simulink library "vmc"  (R2021b)
settings: Solver=VariableStepAuto  StartTime=0.0  StopTime=10.0  RelTol=1e-3
undefined symbols (not defined in the file): AVMC_ACCDeltaTqGradeGn_X_deg, AVMC_ACCDeltaTqIGain4OVRD_X_kph, AVMC_ACCDeltaTqIGain4OVRD_Y_mps2, AVMC_ACCDeltaTqIGain_X_kph, AVMC_ACCDeltaTqIGain_Y_mps2, AVMC_ACCDeltaTqPGain_X_kph, AVMC_ACCDeltaTqPGain_Y_kph, AVMC_ACCGradeofst_X_G, AVMC_ACCGradeofst_Y_pct, AVMC_ACCLoSpdTqLoLim4JP_X_kph, AVMC_ACCLoSpdTqLoLim4JP_Y_deg, AVMC_ACCLoSpdTqLowerLim_X_kph, AVMC_ACCLoSpdTqLowerLim_Y_deg, AVMC_ACCReqAccelGain_X_mps2, AVMC_ACCReqAccelGain_Y_enum, AVMC_ADSPosGFBDeltaTq_X_kph, AVMC_ADSPosGFBDeltaTq_Y_mps2, AVMC_AggressJerkPCT4AT_X_kph, AVMC_AggressJerkPCT_X_kph, AVMC_AggressLimitPCT4AT_X_kph, AVMC_AggressLimitPCT_X_kph, AVMC_DECGradeofst_X_G, AVMC_DECGradeofst_Y_pct, AVMC_DISCDeltaTqIGain_X_kph, AVMC_DISCDeltaTqIGain_Y_mps2, AVMC_DISCDeltaTqPGain_X_kph, AVMC_DISCDeltaTqPGain_Y_kph, AVMC_EPSForceSelect_X_enum, AVMC_EPSForceSelect_Y_enum, AVMC_EPSForceSelectD21_X_enum, AVMC_EPSForceSelectD21_Y_enum, AVMC_ESCRegenOut_X_kph, AVMC_ESCRegenOut_Y_Deg, AVMC_ESCRegenOutEnSpd_X_Deg, AVMC_EstPitchSlopeTs_X_kph, AVMC_GradeCompFlt_X_kph, AVMC_GyroYBandLo_X_Gps, AVMC_HoldResTq_X_kph, AVMC_ISOAccLimit_X_mps, AVMC_ISODecLimit_X_mps, AVMC_ISOJerk_X_mps, AVMC_LatESCRegenOut_X_kph, AVMC_LatESCRegenOut_Y_Deg, AVMC_LongAccDeadZone_X_kph, AVMC_LongAccFiltTsforP2_X_Gps, AVMC_MCPresBaseTq_X_bar, AVMC_MSAPedalOvrd_X_kph, AVMC_MSASpdBand_X_kph, AVMC_MSATqDownEndTq_X_kph, AVMC_MSATqDownTime_X_kph, AVMC_NegZCHoldTq_X_kph, AVMC_OPDDisSlideRate_X_Deg, AVMC_OVRD2ActSR2FCMCMD_X_mps2, AVMC_PedalTqRWhlRatio_X_Nm, AVMC_PedalTqRWhlRatio_Y_gps, AVMC_PedalTqRWhlSlipGain_X_rat, AVMC_PedalTqRWhlSlipGain_Y_kph, AVMC_PedalTqRWhSTRGGain_X_deg, AVMC_PedalTqRWhSTRGGain_Y_kph, AVMC_PosZCHoldTq_X_kph ... (+593)
libraries: hcu_lib x143, simulink x96, tqr x4, $bdroot x1, simulink_extras x1
(part 8 of 17)

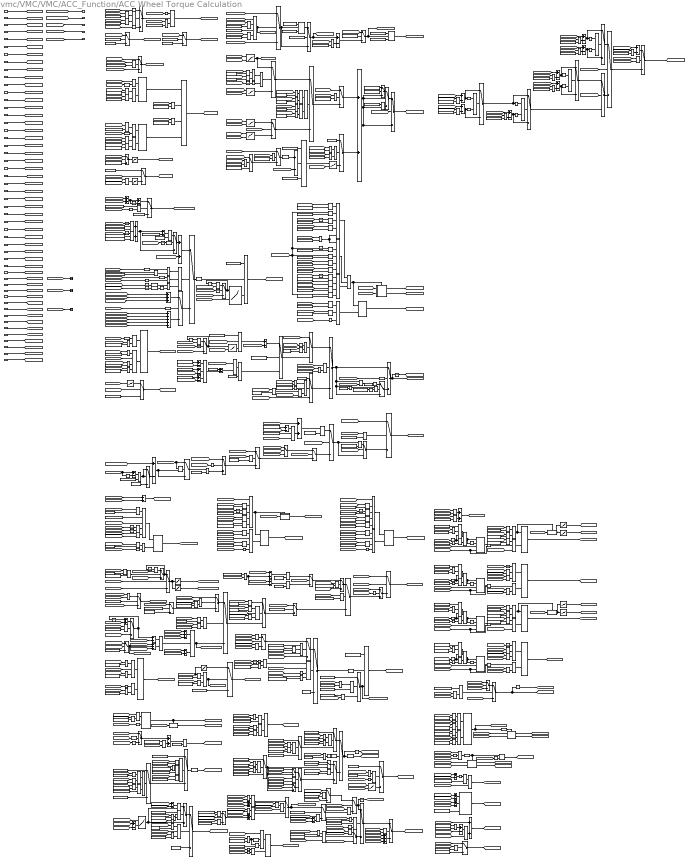
== system vmc/VMC/VMC/ACC_Function/ACC Wheel Torque Calculation ==
  note: HoldTqCalculation
  note: ZeroCrossControl
  note: VehHoldJerkPrevent
  note: ADASWhlTqCalAftHold_ADASWhlTqReq
  note: ADASWhlTqCalBftHold
  note: OriADASWhlTq_ACCLowSpdTq
  note: ACCDeltaTq
  note: GradeHoldResumeAddTq
  note: NegReq_BRgn_TqCompensation
  note: Deceleration Positive Torque Control
  note: Deceleration Torque Control
  note: Deceleration REGEN Torque Control Judgement
  note: Deceleration REGEN Torque Control
  VVMC_LongAcc_Gps : Inport
  VVMC_ActACCRequiredAccel_mps2 : Inport  Port=2
  VVMC_VehicleSpeed_kph : Inport  Port=3
  VVMC_ADASActive_flg : Inport  Port=4
  VTQD_CoordWhlTqDemFr_Nm : Inport  Port=5
  VTQD_CoordWhlTqDemRr_Nm : Inport  Port=6
  VVMC_ACCPedalOvrd_flg : Inport  Port=7
  VVMC_FeatSetSpdForCalcu_kph : Inport  Port=8
  VVMC_FeatArbitrFinal_enum : Inport  Port=9
  VINP_FrTMSpd_rpm : Inport  Port=10
  VINP_RrTMSpd_rpm : Inport  Port=11
  VINP_MCPressure_bar : Inport  Port=12
  VINP_ESCADASSta_enum : Inport  Port=13
  VVMC_FeatReqSpd_kph : Inport  Port=14
  VVMC_MeterIndSpeedForCalcu_kph : Inport  Port=15
  VTQD_SWC2ResUpSta_flg : Inport  Port=16
  VINP_FrntAxlTrqReqBrk_Nm : Inport  Port=17
  VINP_RearAxlTrqReqBrk_Nm : Inport  Port=18
  VTQR_RrTMTqReq_Nm : Inport  Port=19
  VVMC_ACCVehHoldReqRaw_flg : Inport  Port=20
  VVMC_EstSlope_Deg : Inport  Port=21
  VINP_TargetType_enum : Inport  Port=22
  VVMC_SafetyCtrl_flg : Inport  Port=23
  VTQR_FrTMTqReq_Nm : Inport  Port=24
  task_time_s : Inport  Port=25
  VVMC_TotalAvailBrkRgnTq_Nm : Inport  Port=26
  VVMC_AccelTurnHold_flg : Inport  Port=27
  VVMC_ADASACCSta_enum : Inport  Port=28
  VTQD_CreepBaseTqD_Nm : Inport  Port=29
  VVMC_OVRD2ActRampActive_flg : Inport  Port=30
  VINP_ACCRequiredAccel_mps2 : Inport  Port=31
  VTQD_SWC1ResUpSta_flg : Inport  Port=32
  VINP_SWCType_enum : Inport  Port=33
  VVMC_ReqBrkJoin_flg : Inport  Port=34
  VINP_RDCActive_enum : Inport  Port=35
  VINP_BrkSwSta_flg : Inport  Port=36
  VINP_LFWhlRotDir_enum : Inport  Port=37
  VINP_LRWhlRotDir_enum : Inport  Port=38
  VINP_RFWhlRotDir_enum : Inport  Port=39
  VINP_RRWhlRotDir_enum : Inport  Port=40
  VINP_FrEDURealTMTq_Nm : Inport  Port=41
  VINP_FrEDURotateDirction_enum : Inport  Port=42
  VINP_RrEDURealTMTq_Nm : Inport  Port=43
  VINP_RrEDURotateDirction_enum : Inport  Port=44
  VVMC_ACCVehHoldReq_flg : Inport  Port=45
  VVMC_ACCShutOffHold_flg : Inport  Port=46
  VVMC_FrWhlSpdInvalid_flg : Inport  Port=47
  VVMC_RrWhlSpdInvalid_flg : Inport  Port=48
  VVMC_LongAccFrWhl_Gps : Inport  Port=49
  VVMC_LongAccRrWhl_Gps : Inport  Port=50
  " 2" : Constant  Value=ENUM_SWCTYPE_SWC2
  1-D Lookup Table : Lookup_n-D  NumberOfTableDimensions=1  BreakpointsForDimension1=AVMC_ACCDeltaTqGradeGn_X_deg  Table=MVMC_ACCDeltaTqGradeGn_Y_Nm  InternalRulePriority=Speed  RndMeth=Simplest  InputSameDT=on
  AND{,1,4,7..8,10..11,16..18,20..27,31..33,38,41,44,47..49,52..53,55,60,62} (32 alike) : Logic  AllPortsSameDT=off  OutDataTypeStr=boolean
  AND{2,6,12..13,28..30,34,36,39,42,45,50..51,54,56..57,61} (18 alike) : Logic  Inputs=3  AllPortsSameDT=off  OutDataTypeStr=boolean
  AND{14..15,19,35,37,40,43,46} (8 alike) : Logic  Operator=OR  AllPortsSameDT=off  OutDataTypeStr=boolean
  AND3 : Logic  Inputs=4  AllPortsSameDT=off  OutDataTypeStr=boolean
  AND5 : Logic  Inputs=5  AllPortsSameDT=off  OutDataTypeStr=boolean
  AND58 : Logic  Operator=OR  Inputs=3  AllPortsSameDT=off  OutDataTypeStr=boolean
  AND59 : Logic  Operator=OR  Inputs=4  AllPortsSameDT=off  OutDataTypeStr=boolean
  AND9 : Logic  Inputs=4  AllPortsSameDT=off  OutDataTypeStr=boolean
  Abs{,1..8} (9 alike) : Abs
  Add{,3..4,7..8,10..12,14,16,27,30..35,40..46,48} (25 alike) : Sum  Inputs=+-
  Add1 : Sum  Inputs=+++++
  Add{2,5..6,13,15,18..21,23,25..26,28..29,36..39} (18 alike) : Sum
  Add{9,17,22,24} (4 alike) : Sum  Inputs=+++
  Cast To Single{,1..3} (4 alike) : DataTypeConversion  OutDataTypeStr=single
  Constant{1,49,76,113,134} (5 alike) : Constant  Value=KVMC_ACCRgnCtrl2Hold_flg
  Constant10 : Constant  Value=KVMC_ADASWhlTqUpperLim_Nm
  Constant100 : Constant  Value=KVMC_ZeroRgnTqSpdCtrlTime_s
  Constant{4,18..19,22,25,27,29,40,43,45..46,50..53,58,63..64,66..75,81..83,87,89..90,92..94,96,98..99,101..103,109,111..112,114,116..117,119..120,124..125,129..133,136..137,141..144,151..152,154..156,159,163,168,188,191..192,213,215,219,221,228,234} (81 alike) : Constant  Value=ZERO_FLOAT
  Constant104 : Constant  Value=KVMC_HoldAllowZeroTqGrade_deg
  Constant105 : Constant  Value=KVMC_SmallGradeTMRevPrvt_flg
  Constant106 : Constant  Value=KVMC_VehHoldTqIncMinTq_Nm
  Constant{107..108,208,235} (4 alike) : Constant  Value=KVMC_VehHoldTqIncMCP_bar
  Constant11 : Constant  Value=KVMC_ADASWhlTqLowerLim_Nm
  Constant110 : Constant  Value=KVMC_NegReqEnSpd_kph
  Constant115 : Constant  Value=KVMC_TMRevPrvtTqAddEveryTT_flg
  Constant118 : Constant  Value=KVMC_ACCLoSpdFollowBRgnSW_flg
  Constant12 : Constant  Value=KVMC_AccDevLowLim_mps2
  Constant121 : Constant  Value=KVMC_VHJerkPrvt_flg
  Constant122 : Constant  Value=KVMC_VehHoldDecSR_Nm
  Constant123 : Constant  Value=ENUM_FEATARBITRSTA_DISC
  Constant126 : Constant  Value=KVMC_ADASWhlTqLowerLim_Nm
  Constant127 : Constant  Value=KVMC_VHJerkPrvt_flg
  Constant{41,44,47..48,78..79,91,128,149} (9 alike) : Constant  Value=KVMC_ZeroRgnTqSpd_kph
  Constant13 : Constant  Value=KVMC_AccDevUpLim_mps2
  Constant135 : Constant  Value=KVMC_NegReqDeltaTqGain_rat
  Constant138 : Constant  Value=KVMC_ReqAccelLimitSW_flg
  Constant139 : Constant  Value=KVMC_MaxReqAccel_mps2
  Constant14 : Constant  Value=KVMC_ACCSpdDevUpLim_kph
  Constant140 : Constant  Value=KVMC_MinReqAccel_mps2
  Constant145 : Constant  Value=ENUM_CANRDCACTSTA_EXITIMMEDIATELY
  Constant146 : Constant  Value=KVMC_ADASWhlTqUpperLim_Nm
  Constant147 : Constant  Value=ENUM_CANRDCACTSTA_NOREQUEST
  Constant148 : Constant  Value=KVMC_VHTMSpdCtrlChkTMDir_flg
  Constant15 : Constant  Value=KVMC_ACCSpdDevLowLim_kph
  Constant150 : Constant  Value=KVMC_VHTMSpdCtrlSR_raw32
  Constant153 : Constant  Value=KVMC_ZeroCrossTestSW_flg
  Constant157 : Constant  Value=KTQD_FrTMTotalGearRatio_gain
  Constant158 : Constant  Value=KTQD_RrTMTotalGearRatio_gain
  Constant16 : Constant  Value=ENUM_FEATARBITRSTA_ACC
  Constant160 : Constant  Value=KVMC_VHTMSpdCtrlChkTMDir_flg
  Constant{161..162,171..172,189..190,193..194} (8 alike) : Constant  Value=KVMC_ZCChkRealWhlTqSW_flg
  Constant164 : Constant  Value=KVMC_ESCSSMCPThres_bar
  Constant{165,169..170,173..174,176,184,203..205} (10 alike) : Constant  Value=ENUM_WheelRotDir_BACKWARD
  Constant166 : Constant  Value=ENUM_ESCADASSTA_VEHASTANDSTILL
  Constant167 : Constant  Value=KVMC_StandstillTqRamp2ZeroSlope_Nmps
  Constant{17,211,224,226,232} (5 alike) : Constant  Value=ENUM_ADASACCSTA_ACTIVE
  Constant{175,177..178,181,197,206} (6 alike) : Constant  Value=ENUM_WheelRotDir_FORWARD
  Constant{179..180,182..183,185..187,198,200} (9 alike) : Constant  Value=ENUM_WheelRotDir_STANDSTILL
  Constant195 : Constant  Value=ENUM_TMROTATEDIRECTACT_STOP
  Constant196 : Constant  Value=ENUM_TMROTATEDIRECTACT_REVERSE
  Constant199 : Constant  Value=KVMC_HoldAdd2GradeGn_flg
  Constant{2,7..8,20} (4 alike) : Constant  Value=KVMC_HillUpResetTMSpd_rpm
  Constant201 : Constant  Value=KVMC_VHTMSpdCtrlChkTMDir_flg
  Constant202 : Constant  Value=ENUM_TMROTATEDIRECTACT_STOP
  Constant207 : Constant  Value=KVMC_IgnrAvailBrgnSpd_kph
  Constant209 : Constant  Value=KVMC_HoldTqCalSpd1_kph
  Constant21 : Constant  Value=ENUM_FEATARBITRSTA_DISC
  Constant{9,210,229,237..243,245} (11 alike) : Constant  Value=KVMC_GravityValue_mps2
  Constant212 : Constant  Value=KVMC_HoldTqCalDeltaAccThres_Gps
  Constant214 : Constant  Value=KVMC_HoldTqCtrlTargetGx_mps2
  Constant{216..218,223} (4 alike) : Constant  Value=KVMC_HoldTqCalTest_flg
  Constant220 : Constant  Value=MINUSONE_FLOAT
  Constant222 : Constant  Value=KVMC_AccTurnHoldTqDecSR_Nmps
  Constant225 : Constant  Value=KVMC_HoldTqCalSpd1_kph
  Constant227 : Constant  Value=KVMC_HoldGradeOnlyInc_flg
  Constant23 : Constant  Value=KVMC_OVRDResSmoothTest_SW
  Constant230 : Constant  Value=KVMC_HoldTqAddDisDec_mps2
  Constant231 : Constant  Value=KVMC_HoldResTqDisSpd_kph
  Constant233 : Constant  Value=KVMC_HoldResTqDisDeltaAcc_mps2
  Constant236 : Constant  Value=KVMC_CompareFrRrLongAcl_flg
  Constant24 : Constant  Value=KVMC_OVRD2ActRgnTarget_Nm
  Constant26 : Constant  Value=KVMC_AddBRegen2ACCLoop_flg
  Constant28 : Constant  Value=KVMC_HoldTqCtrlGradeThres_deg
  Constant3 : Constant  Value=ENUM_ESCADASSTA_VEHASTANDSTILL
  Constant30 : Constant  Value=KVMC_TqSafetyCtrl_flg
  Constant31 : Constant  Value=KVMC_ACCResUpEnAccCMD_mps2
  Constant32 : Constant  Value=KVMC_HoldTqCtrlSourceSW_flg
  Constant33 : Constant  Value=KVMC_SoftUphillTqIncSR_Nm
  Constant34 : Constant  Value=KVMC_ADASWhlTqUpperLim_Nm
  Constant35 : Constant  Value=KVMC_NegReqZeroPosTq_flg
  Constant{6,36..37,62,77,80,88,97} (8 alike) : Constant  Value=KVMC_CutOffNegTqSpd_kph
  Constant38 : Constant  Value=KTQR_FrTMGearEff_c
  Constant39 : Constant  Value=KVMC_ACCDeltaTqFollowADSCmd_flg
  Constant42 : Constant  Value=KTQD_FrTMTotalGearRatio_gain
  Constant5 : Constant  Value=KVMC_AddBRegen2ACCLoop_flg
  Constant54 : Constant  Value=KVMC_NegReqSwEnSpd_kph
  Constant55 : Constant  Value=KVMC_NegReqSwEnSlope_Deg
  Constant56 : Constant  Value=KVMC_ACCResUpEnGrade_Deg
  Constant57 : Constant  Value=ENUM_TARGETTYPE_NONE
  Constant59 : Constant  Value=KVMC_TqMCPRelFactor_Nm
  Constant60 : Constant  Value=ENUM_FEATARBITRSTA_ACC
  Constant61 : Constant  Value=ENUM_FEATARBITRSTA_ACC
  Constant65 : Constant  Value=KVMC_TMRevSpdThres_rpm
  Constant84 : Constant  Value=KTQD_RrTMTotalGearRatio_gain
  Constant85 : Constant  Value=KTQR_RrTMGearEff_c
  Constant86 : Constant  Value=KVMC_OVRDResTqDec4Smooth_Nm
  Constant95 : Constant  Value=KVMC_TMRevSpdPassThres_rpm
  Data Type Conversion1 : DataTypeConversion  OutDataTypeStr=single
  Detect Change : simulink/Logic and Bit Operations/Detect Change  vinit=0  OutDataTypeStr=boolean
  Detect Change1 : simulink/Logic and Bit Operations/Detect Change  vinit=0  OutDataTypeStr=boolean
  Detect Decrease{,1..3} (4 alike) : simulink/Logic and Bit Operations/Detect Decrease  vinit=0.0  OutDataTypeStr=boolean
  Detect Increase{,1..8} (9 alike) : simulink/Logic and Bit Operations/Detect Increase  vinit=0.0  OutDataTypeStr=boolean
  Divide : Product  Inputs=*/*
  Divide1 : Product  Inputs=***
  Divide{2,4,6..11} (8 alike) : Product  Inputs=**
  Divide3 : Product  Inputs=*/*
  Divide5 : Product  Inputs=***
  Equal : RelationalOperator  Operator===  OutDataTypeStr=boolean  RndMeth=Simplest
  Equal1 : RelationalOperator  Operator=<=  OutDataTypeStr=boolean  RndMeth=Simplest
  Equal10 : RelationalOperator  Operator===  OutDataTypeStr=boolean  RndMeth=Simplest
  Equal{4,6,8,11} (4 alike) : RelationalOperator  Operator=<  OutDataTypeStr=boolean  RndMeth=Simplest
  Equal{7,9,12,14} (4 alike) : RelationalOperator  Operator=>  OutDataTypeStr=boolean  RndMeth=Simplest
  Equal13 : RelationalOperator  Operator=<=  OutDataTypeStr=boolean  RndMeth=Simplest
  Equal2 : RelationalOperator  Operator=~=  OutDataTypeStr=boolean  RndMeth=Simplest
  Equal3 : RelationalOperator  OutDataTypeStr=boolean  RndMeth=Simplest
  Equal5 : RelationalOperator  OutDataTypeStr=boolean  RndMeth=Simplest
  Logical Operator : Logic  Inputs=4  AllPortsSameDT=off  OutDataTypeStr=boolean
  Logical Operator1 : Logic  Operator=OR  Inputs=3  AllPortsSameDT=off  OutDataTypeStr=boolean
  Logical Operator{2,4,6,8} (4 alike) : Logic  Inputs=5  AllPortsSameDT=off  OutDataTypeStr=boolean
  Logical Operator3 : Logic  Operator=OR  Inputs=3  AllPortsSameDT=off  OutDataTypeStr=boolean
  Logical Operator5 : Logic  AllPortsSameDT=off  OutDataTypeStr=boolean
  Logical Operator7 : Logic  Operator=OR  Inputs=4  AllPortsSameDT=off  OutDataTypeStr=boolean
  Logical Operator9 : Logic  Operator=OR  Inputs=4  AllPortsSameDT=off  OutDataTypeStr=boolean
  MVMC_ACCDeltaTqIGain4OVRD_Z_Nm : Lookup_n-D  BreakpointsForDimension1=AVMC_ACCDeltaTqIGain4OVRD_Y_mps2  BreakpointsForDimension2=AVMC_ACCDeltaTqIGain4OVRD_X_kph  Table=MVMC_ACCDeltaTqIGain4OVRD_Z_Nm  InternalRulePriority=Speed  RndMeth=Simplest  InputSameDT=on
      settings: InputPortMap=u0,u1
  MVMC_ACCDeltaTqIGain_Z_Nm : Lookup_n-D  BreakpointsForDimension1=AVMC_ACCDeltaTqIGain_Y_mps2  BreakpointsForDimension2=AVMC_ACCDeltaTqIGain_X_kph  Table=MVMC_ACCDeltaTqIGain_Z_Nm  InternalRulePriority=Speed  RndMeth=Simplest  InputSameDT=on
      settings: InputPortMap=u0,u1
  MVMC_ACCDeltaTqPGain_Z_Nm1 : Lookup_n-D  BreakpointsForDimension1=AVMC_ACCDeltaTqPGain_Y_kph  BreakpointsForDimension2=AVMC_ACCDeltaTqPGain_X_kph  Table=MVMC_ACCDeltaTqPGain_Z_Nm  InternalRulePriority=Speed  RndMeth=Simplest  InputSameDT=on
      settings: InputPortMap=u0,u1
  MVMC_ACCLoSpdTqLoLim4JP_Z_Nm : Lookup_n-D  BreakpointsForDimension1=AVMC_ACCLoSpdTqLoLim4JP_Y_deg  BreakpointsForDimension2=AVMC_ACCLoSpdTqLoLim4JP_X_kph  Table=MVMC_ACCLoSpdTqLoLim4JP_Z_Nm  InternalRulePriority=Speed  RndMeth=Simplest  InputSameDT=on
      settings: InputPortMap=u0,u1
  MVMC_ACCLoSpdTqLowerLim_Z_Nm : Lookup_n-D  BreakpointsForDimension1=AVMC_ACCLoSpdTqLowerLim_Y_deg  BreakpointsForDimension2=AVMC_ACCLoSpdTqLowerLim_X_kph  Table=MVMC_ACCLoSpdTqLowerLim_Z_Nm  InternalRulePriority=Speed  RndMeth=Simplest  InputSameDT=on
      settings: InputPortMap=u0,u1
  MVMC_ADSPosGFBDeltaTq_Z_Nm1 : Lookup_n-D  BreakpointsForDimension1=AVMC_ADSPosGFBDeltaTq_Y_mps2  BreakpointsForDimension2=AVMC_ADSPosGFBDeltaTq_X_kph  Table=MVMC_ADSPosGFBDeltaTq_Z_Nm  InternalRulePriority=Speed  RndMeth=Simplest  InputSameDT=on
      settings: InputPortMap=u0,u1
  MVMC_DISCDeltaTqIGain_Z_Nm : Lookup_n-D  BreakpointsForDimension1=AVMC_DISCDeltaTqIGain_Y_mps2  BreakpointsForDimension2=AVMC_DISCDeltaTqIGain_X_kph  Table=MVMC_DISCDeltaTqIGain_Z_Nm  InternalRulePriority=Speed  RndMeth=Simplest  InputSameDT=on
      settings: InputPortMap=u0,u1
  MVMC_HoldResTq_Y_Nm : Lookup_n-D  NumberOfTableDimensions=1  BreakpointsForDimension1=AVMC_HoldResTq_X_kph  Table=MVMC_HoldResTq_Y_Nm  InternalRulePriority=Speed  RndMeth=Simplest  InputSameDT=on
  MVMC_MCPresBaseTq_Y_Nm : Lookup_n-D  NumberOfTableDimensions=1  BreakpointsForDimension1=AVMC_MCPresBaseTq_X_bar  Table=MVMC_MCPresBaseTq_Y_Nm  InternalRulePriority=Speed  RndMeth=Simplest  InputSameDT=on
  MVMC_NegZCHoldTq_Y_Nm : Lookup_n-D  NumberOfTableDimensions=1  BreakpointsForDimension1=AVMC_NegZCHoldTq_X_kph  Table=MVMC_NegZCHoldTq_Y_Nm  InternalRulePriority=Speed  RndMeth=Simplest  InputSameDT=on
  MVMC_PosZCHoldTq_Y_Nm : Lookup_n-D  NumberOfTableDimensions=1  BreakpointsForDimension1=AVMC_PosZCHoldTq_X_kph  Table=MVMC_PosZCHoldTq_Y_Nm  InternalRulePriority=Speed  RndMeth=Simplest  InputSameDT=on
  MVMC_TMRevPrvtTq4JP_Z_Nm : Lookup_n-D  BreakpointsForDimension1=AVMC_TMRevPrvtTq4JP_Y_enum  BreakpointsForDimension2=AVMC_TMRevPrvtTq4JP_X_rpm  Table=MVMC_TMRevPrvtTq4JP_Z_Nm  InternalRulePriority=Speed  RndMeth=Simplest  InputSameDT=on
      settings: InputPortMap=u0,u1
  MVMC_TMRevPrvtTq_Y_Nm : Lookup_n-D  NumberOfTableDimensions=1  BreakpointsForDimension1=AVMC_TMRevPrvtTq_X_rpm  Table=MVMC_TMRevPrvtTq_Y_Nm  InternalRulePriority=Speed  RndMeth=Simplest  InputSameDT=on
  MVMC_TMSpdBaseTq_Y_Nm : Lookup_n-D  NumberOfTableDimensions=1  BreakpointsForDimension1=AVMC_TMSpdBaseTq_X_rpm  Table=MVMC_TMSpdBaseTq_Y_Nm  InternalRulePriority=Speed  RndMeth=Simplest  InputSameDT=on
  MVMC_VHTMSpdCtrl_Z_Nm : Lookup_n-D  BreakpointsForDimension1=AVMC_VHTMSpdCtrl_Y_enum  BreakpointsForDimension2=AVMC_VHTMSpdCtrl_X_rpm  Table=MVMC_VHTMSpdCtrl_Z_Nm  InternalRulePriority=Speed  RndMeth=Simplest  InputSameDT=on
      settings: InputPortMap=u0,u1
  MVMC_VehHoldTqIncGain_Y_Nm : Lookup_n-D  NumberOfTableDimensions=1  BreakpointsForDimension1=AVMC_VehHoldTqIncGain_X_deg  Table=MVMC_VehHoldTqIncGain_Y_Nm  InternalRulePriority=Speed  RndMeth=Simplest  InputSameDT=on
  MVMC_ZCWaitTimeNeg_Y_s : Lookup_n-D  NumberOfTableDimensions=1  BreakpointsForDimension1=AVMC_ZCWaitTimeNeg_X_kph  Table=MVMC_ZCWaitTimeNeg_Y_s  InternalRulePriority=Speed  RndMeth=Simplest  InputSameDT=on
  MVMC_ZCWaitTimePos_Y_s : Lookup_n-D  NumberOfTableDimensions=1  BreakpointsForDimension1=AVMC_ZCWaitTimePos_X_kph  Table=MVMC_ZCWaitTimePos_Y_s  InternalRulePriority=Speed  RndMeth=Simplest  InputSameDT=on
  Max{,1,4,6..8,10} (7 alike) : MinMax  Function=max  Inputs=2
  Max{2..3,5,9,12} (5 alike) : MinMax  Inputs=2
  Min{,1,3,6..8,13..14} (8 alike) : MinMax  Inputs=2
  Min{2,4..5,9..12,15..17} (10 alike) : MinMax  Function=max  Inputs=2
  NOT{,1..33} (34 alike) : Logic  Operator=NOT  AllPortsSameDT=off  OutDataTypeStr=boolean
  OR{,1,4,6..10,12,16..20} (14 alike) : Logic  Operator=OR  AllPortsSameDT=off  OutDataTypeStr=boolean
  OR{2..3,11,13} (4 alike) : Logic  Operator=OR  Inputs=3  AllPortsSameDT=off  OutDataTypeStr=boolean
  OR14 : Logic  AllPortsSameDT=off  OutDataTypeStr=boolean
  OR15 : Logic  AllPortsSameDT=off  OutDataTypeStr=boolean
  OR21 : Logic  AllPortsSameDT=off  OutDataTypeStr=boolean
  OR5 : Logic  Inputs=4  AllPortsSameDT=off  OutDataTypeStr=boolean
  Product{1,3..12} (11 alike) : Product
  Product2 : Product  Inputs=*/
  Relational Operator{,2..4,7,13,16,27,32..33,38,44,47,58..63,66,68,76,80,85,100..101,106,111..113,115,117} (32 alike) : RelationalOperator  Operator=>  OutDataTypeStr=boolean  RndMeth=Simplest
  Relational Operator{1,20,34,40,51,57,65,67,77,107,109,121,124..127} (16 alike) : RelationalOperator  Operator=<=  OutDataTypeStr=boolean  RndMeth=Simplest
  Relational Operator{8,10,12,24..25,29,36..37,39,42..43,48,53,70,72,75,78..79,82..83,110,119,122} (23 alike) : RelationalOperator  OutDataTypeStr=boolean  RndMeth=Simplest
  Relational Operator{5..6,17,19,55..56,64,69,73,86..97,102..105,114,118} (27 alike) : RelationalOperator  Operator===  OutDataTypeStr=boolean  RndMeth=Simplest
  Relational Operator{9,11,14..15,21..23,26,28,30..31,35,41,45..46,49..50,52,54,71,74,81,84,98..99,108,123} (27 alike) : RelationalOperator  Operator=<  OutDataTypeStr=boolean  RndMeth=Simplest
  Relational Operator116 : RelationalOperator  Operator=~=  OutDataTypeStr=boolean  RndMeth=Simplest
  Relational Operator120 : RelationalOperator  Operator=~=  OutDataTypeStr=boolean  RndMeth=Simplest
  Relational Operator18 : RelationalOperator  Operator=~=  OutDataTypeStr=boolean  RndMeth=Simplest
  Relay : Relay  OnSwitchValue=KVMC_ACCTq2ZeroEnMCPress2_bar  OffSwitchValue=KVMC_ACCTq2ZeroDisMCPress2_bar  OutDataTypeStr=boolean
  Relay1 : Relay  OnSwitchValue=KVMC_ACCTq2ZeroEnMCPress_bar  OffSwitchValue=KVMC_ACCTq2ZeroDisMCPress_bar  OutDataTypeStr=boolean
  SR_Latch{,1..16} (17 alike) : hcu_lib/Basic_Blocks/SR_Latch
  Saturation Dynamic{1..7} (7 alike) : simulink/Discontinuities/Saturation Dynamic  OutMin=[]  OutMax=[]  OutDataTypeStr=Inherit: Same as second input  OutDataType=fixdt(1, 16)  OutScaling=2^-10  DoSatur=off
  Switch{,1..89} (90 alike) : Switch  Criteria=u2 > Threshold
  Terminator : Terminator
  Terminator1 : Terminator
  Terminator2 : Terminator
  Timer{1..4} (4 alike) : hcu_lib/Basic_Blocks/Timer
  Triggered Subsystem : Subsystem  TreatAsAtomicUnit=on
  Triggered Subsystem1 : Subsystem  TreatAsAtomicUnit=on
  Triggered Subsystem2 : Subsystem  TreatAsAtomicUnit=on
  Triggered Subsystem3 : $bdroot/VMC/VMC/ACC_Function/ACC Wheel Torque Calculation/Triggered Subsystem2  SystemSampleTime=-1  VariantActivationTime=update diagram  Latency=0  AutoFrameSizeCalculation=off
  Triggered Subsystem4 : Subsystem  TreatAsAtomicUnit=on
  Triggered Subsystem5 : Subsystem  TreatAsAtomicUnit=on
  Triggered Subsystem6 : Subsystem  TreatAsAtomicUnit=on
  Unit Delay{,1..33} (34 alike) : UnitDelay  SampleTime=-1  HasFrameUpgradeWarning=on
  divide : hcu_lib/Basic_Blocks/divide
  ic0 : UnitDelay  SampleTime=-1  HasFrameUpgradeWarning=on
  u2 > 0 : Switch  Criteria=u2 > Threshold
  u2 > 0 (1) : Switch  Criteria=u2 > Threshold
  u2 > 0 (3) : Switch  Criteria=u2 > Threshold
  u2 > 0 (4) : Switch  Criteria=u2 > Threshold
  VVMC_ADASWhlTqCal_Nm : Outport
  VVMC_ADASNegReq_flg : Outport  Port=2
  VVMC_ACCLowSpdTqCtrl_flg : Outport  Port=3
  VVMC_ACCWhlTqLowerLim_Nm : Outport  Port=4
  VVMC_RrWhlStandstill_flg : Outport  Port=5
  wires:
  [VVMC_ADASActive_flg] -> Logical Operator8/1
  [VVMC_ADASActive_flg] -> Logical Operator6/1
  VINP_SWCType_enum/1 -> [VINP_SWCType_enum]
  [VTQD_SWC1ResUpSta_flg] -> Switch2/3
  VTQD_SWC1ResUpSta_flg/1 -> [VTQD_SWC1ResUpSta_flg]
  [VTQD_SWC2ResUpSta_flg] -> Switch2/1
  Relational Operator56/1 -> Switch2/2
  " 2"/1 -> Relational Operator56/2
  [VINP_SWCType_enum] -> Relational Operator56/1
  MVMC_ADSPosGFBDeltaTq_Z_Nm1/1 -> Switch40/3  "VVMC_ADSPosGFBPCTDeltaTq_Nm"
  [VVMC_VehicleSpeed_kph] -> MVMC_ADSPosGFBDeltaTq_Z_Nm1/2
  [VVMC_ActAccDev_mps2] -> MVMC_ADSPosGFBDeltaTq_Z_Nm1/1
  AND18/1 -> AND15/1
  Switch40/1 -> Switch34/1
  [VVMC_LongAcc_Gps] -> Equal11/1
  [VVMC_ActACCRequiredAccel_mps2] -> Equal12/1
  Constant71/1 -> Equal12/2
  Constant68/1 -> Equal11/2
  Equal11/1 -> AND18/1
  Equal12/1 -> AND18/2
  [VVMC_DISCDeltaTqIGain_Nm] -> Switch33/1
  Switch26/1 -> Switch34/3
  [VVMC_VehicleSpeed_kph] -> MVMC_ACCDeltaTqIGain4OVRD_Z_Nm/2
  MVMC_ACCDeltaTqIGain4OVRD_Z_Nm/1 -> Switch26/1  "VVMC_ACCDeltaTqIGain4OVRD_Nm"
  [VVMC_OVRDAccCtrl_flg] -> Switch26/2
  [VINP_ACCRequiredAccel_mps2] -> Switch9/1
  [VVMC_ActACCRequiredAccel_mps2] -> Switch9/3
  AND9/1 -> Switch9/2, [VVMC_OVRDAccCtrl_flg]  "VVMC_OVRDAccCtrl_flg"
  Relational Operator27/1 -> AND9/4
  Constant24/1 -> Relational Operator27/2
  [VVMC_LastADASWhlTqCal_Nm] -> Relational Operator27/1
  Constant23/1 -> AND9/3
  Relational Operator1/1 -> AND9/2
  Constant18/1 -> Relational Operator1/2
  [VINP_ACCRequiredAccel_mps2] -> Relational Operator1/1
  [VVMC_OVRD2ActRampActive_flg] -> AND9/1
  VINP_ACCRequiredAccel_mps2/1 -> [VINP_ACCRequiredAccel_mps2]
  VVMC_OVRD2ActRampActive_flg/1 -> [VVMC_OVRD2ActRampActive_flg]
  Min5/1 -> Switch36/1
  NOT8/1 -> OR7/2
  Add23/1 -> Min5/1
  Constant94/1 -> Min5/2
  Constant86/1 -> Add23/2
  Detect Decrease1/1 -> Switch36/2
  Unit Delay13/1 -> Detect Decrease1/1
  [VVMC_ACCPedalOvrd_flg] -> Unit Delay13/1
  [VVMC_ADASActive_flg] -> OR5/2
  Relational Operator61/1 -> OR8/2
  Relational Operator39/1 -> Logical Operator6/2
  [VVMC_LastADASWhlTqCal_Nm] -> Relational Operator13/1
  OR8/1 -> Switch30/2
  [VVMC_VehicleSpeed_kph] -> Relational Operator61/1
  Constant44/1 -> Relational Operator61/2
  Unit Delay8/1 -> Relational Operator36/1
  [VVMC_ACCVehHoldReqRaw_flg] -> NOT3/1
  [VVMC_ActACCRequiredAccel_mps2] -> Relational Operator37/1
  Relational Operator52/1 -> AND6/1
  Constant30/1 -> AND12/1
  Relational Operator53/1 -> OR4/2
  Constant103/1 -> Relational Operator51/2
  [VVMC_ACCLowSpdFollowESCTq_flg] -> OR8/1
  Relational Operator73/1 -> OR6/2
  Equal10/1 -> Switch41/2
  [VVMC_VehicleSpeed_kph] -> Relational Operator38/1
  Constant166/1 -> Equal10/2
  Relational Operator19/1 -> AND12/2
  Switch11/1 -> [VVMC_ADASWhlTqCalAftHold_Nm]  "VVMC_ADASWhlTqCalAftHold_Nm"
  NOT3/1 -> Switch7/2
  Constant10/1 -> Saturation Dynamic3/1
  Constant87/1 -> Relational Operator37/2
  Constant88/1 -> Relational Operator38/2
  [VVMC_ActACCRequiredAccel_mps2] -> Relational Operator35/1
  Constant81/1 -> Relational Operator35/2
  Constant80/1 -> Relational Operator34/2
  OR4/1 -> SR_Latch2/2
  [VVMC_SafetyCtrl_flg] -> AND12/3
  [VVMC_FeatArbitrFinal_enum] -> Relational Operator19/1
  [VVMC_MCPreBaseTqEn_flg] -> Switch11/2
  Relational Operator36/1 -> Logical Operator6/3
  [VVMC_LastADASWhlTqCal_Nm] -> Relational Operator39/1
  Switch55/1 -> [VVMC_ADASWhlTqCal_Nm], ic0/1  "VVMC_ADASWhlTqCal_Nm"
  SR_Latch3/1 -> [VVMC_RgnProhibited_flg]  "VVMC_RgnProhibited_flg"
  [VVMC_ActACCRequiredAccel_mps2] -> Unit Delay8/1
  [VVMC_VehicleSpeed_kph] -> Relational Operator34/1
  OR5/1 -> Switch5/2
  OR6/1 -> OR5/1
  Equal4/1 -> AND29/3
  NOT7/1 -> Logical Operator7/4
  u2 > 0 (4)/1 -> u2 > 0 (3)/1  "VVMC_ADASWhlTqCalAftSafety_Nm"
  [VVMC_LastADASWhlTqCal_Nm] -> u2 > 0 (4)/2
  Logical Operator7/1 -> SR_Latch3/2
  Relational Operator38/1 -> Logical Operator7/1
  [VVMC_TotalAvailBrkRgnTq_Nm] -> Max6/2
  [VINP_MCPressure_bar] -> Relational Operator53/1
  Constant90/1 -> Relational Operator39/2
  [VVMC_ACCPedalOvrd_flg] -> Unit Delay4/1
  u2 > 0 (3)/1 -> Switch5/1
  Switch5/1 -> Cast To Single3/1
  [VVMC_ADASWhlTqCalBftHold_Nm] -> Switch7/1
  Constant11/1 -> Max6/1
  [VVMC_LastADASWhlTqCal_Nm] -> Add22/3
  [VVMC_ADASActive_flg] -> NOT7/1
  Constant168/1 -> Max8/2
  Switch45/1 -> Switch30/3
  Relational Operator34/1 -> Logical Operator6/5
  Add21/1 -> Max8/1
  [VVMC_LastADASWhlTqCal_Nm] -> Add21/1
  Constant17/1 -> Relational Operator73/2
  [VVMC_ADASACCSta_enum] -> Relational Operator73/1
  Constant167/1 -> Divide7/1
  NOT4/1 -> OR6/1
  Relational Operator35/1 -> Logical Operator6/4
  Constant61/1 -> Relational Operator19/2
  [VVMC_LastADASWhlTqCal_Nm] -> Add17/1
  [VINP_ESCADASSta_enum] -> Equal10/1
  Add17/1 -> Max9/2
  Switch41/1 -> Switch7/3  "VVMC_ADASWhlTqCalVehHold_Nm"
  Switch31/1 -> [VVMC_UphillTqIncSRFinal_Nm], Add17/2
  Relational Operator13/1 -> AND6/3
  Switch7/1 -> Switch11/3
  Switch30/1 -> Switch28/1
  Constant104/1 -> Equal4/2
  Relational Operator51/1 -> AND7/1
  Constant33/1 -> Switch31/3
  [VVMC_HoldNoMCP_flg] -> Switch31/2
  [VVMC_EstSlope_Deg] -> Equal4/1
  [VINP_MCPressure_bar] -> Relational Operator52/1
  AND12/1 -> u2 > 0 (3)/2
  Switch47/1 -> Saturation Dynamic3/3, [VVMC_ACCWhlTqLowerLim_Nm]
  Constant122/1 -> Add19/2
  [VVMC_ACCVehHoldReqRaw_flg] -> NOT6/1
  AND29/1 -> Switch39/2
  Constant82/1 -> Relational Operator36/2
  Relational Operator37/1 -> Logical Operator7/3
  NOT6/1 -> OR4/1
  Constant108/1 -> Relational Operator53/2
  [VVMC_VehHoldCtrlTq_Nm] -> Add25/2
  Switch28/1 -> Switch39/3
  Cast To Single3/1 -> Saturation Dynamic3/2
  SR_Latch2/1 -> [VVMC_HoldNoMCP_flg]  "VVMC_HoldNoMCP_flg"
  Unit Delay4/1 -> NOT4/1
  Constant107/1 -> Relational Operator52/2
  Constant106/1 -> Relational Operator13/2
  AND6/1 -> SR_Latch2/1
  [task_time_s] -> Divide7/2
  Add19/1 -> Saturation Dynamic2/3
  [VVMC_LastADASWhlTqCal_Nm] -> Add19/1
  Switch39/1 -> Switch48/3
  Add22/1 -> Saturation Dynamic2/1
  Constant74/1 -> Switch5/3
  [VVMC_AccelTurnHold_flg] -> AND29/2
  Logical Operator6/1 -> SR_Latch3/1
  [VVMC_ACCVehHoldReqRaw_flg] -> AND6/2
  Switch36/1 -> Add5/1
  [VVMC_OriADASWhlTq_Nm] -> Triggered Subsystem1/1(In1)
  OR7/1 -> SR_Latch5/2
  Logical Operator9/1 -> SR_Latch4/2
  [VVMC_ACCDeltaAccel_mps2] -> Relational Operator58/1
  [VVMC_ActACCRequiredAccel_mps2] -> Relational Operator54/1
  Relational Operator54/1 -> AND5/1
  Constant120/1 -> Relational Operator54/2
  [VVMC_ACCLowSpdTqCtrl_flg] -> NOT8/1
  Relational Operator58/1 -> OR7/1
  Constant109/1 -> Relational Operator58/2
  VTQD_CreepBaseTqD_Nm/1 -> [VTQD_CreepBaseTqD_Nm]
  Switch20/1 -> Switch18/1  "VVMC_ACCLowSpdTqAftFollowESC_Nm"
  Relational Operator50/1 -> AND16/1
  [VVMC_ACCLowSpdFollowESCTq_flg] -> Switch20/2
  [VVMC_TotalESCBRgnReq_Nm] -> Switch20/1
  Max4/1 -> Min1/1
  SR_Latch5/1 -> [VVMC_ACCLowSpdFollowESCTq_flg]  "VVMC_ACCLowSpdFollowESCTq_flg"
  [VVMC_ACCLowSpdTqCtrl_flg] -> AND5/3
  AND5/1 -> SR_Latch5/1
  Relational Operator48/1 -> AND5/5
  Relational Operator46/1 -> AND5/4
  [VVMC_ACCLowSpdTq_Nm] -> Relational Operator48/1
  [VVMC_TotalESCBRgnReq_Nm] -> Relational Operator48/2
  Unit Delay11/1 -> Relational Operator46/2
  [VVMC_TotalESCBRgnReq_Nm] -> Unit Delay11/1
  Unit Delay10/1 -> Relational Operator46/1
  [VVMC_ACCLowSpdTq_Nm] -> Unit Delay10/1
  Add2/1 -> [VVMC_TotalESCBRgnReq_Nm]
  [VINP_FrntAxlTrqReqBrk_Nm] -> Add2/1
  [VINP_RearAxlTrqReqBrk_Nm] -> Add2/2
  [VVMC_ADASNegReq_flg] -> AND14/2
  NOT5/1 -> Switch16/2
  Switch16/1 -> Switch19/3
  [VVMC_ADASNegReq_flg] -> NOT5/1
  Switch37/1 -> Add7/1, [VVMC_ACCReqAclAftLim_mps2]
  Constant138/1 -> Switch37/2
  Constant140/1 -> Saturation Dynamic1/3
  Switch9/1 -> Switch37/3, Saturation Dynamic1/2
  Constant139/1 -> Saturation Dynamic1/1
  Saturation Dynamic1/1 -> Switch37/1
  Switch8/1 -> Switch6/3
  Detect Decrease3/1 -> AND/1
  Unit Delay2/1 -> Detect Change/1
  [VVMC_FeatArbitrFinal_enum] -> Unit Delay2/1
  [VVMC_ACCPedalOvrd_flg] -> Unit Delay1/1
  NOT/1 -> AND/2
  Detect Change/1 -> NOT/1
  Unit Delay1/1 -> Detect Decrease3/1
  VVMC_ADASACCSta_enum/1 -> [VVMC_ADASACCSta_enum]
  VVMC_AccelTurnHold_flg/1 -> [VVMC_AccelTurnHold_flg]
  VVMC_TotalAvailBrkRgnTq_Nm/1 -> [VVMC_TotalAvailBrkRgnTq_Nm]
  Relational Operator7/1 -> AND3/2
  Detect Increase2/1 -> AND4/2
  Switch19/1 -> Switch18/3  "VVMC_ACCTqNegReqNotLowSpd_Nm"
  Constant132/1 -> Equal9/2
  [VVMC_ACCDeltaAccel_mps2] -> Equal9/1
  Equal9/1 -> AND20/2
  AND20/1 -> AND19/2
  Equal8/1 -> AND20/1
  [VVMC_ActACCRequiredAccel_mps2] -> Equal8/1
  Constant131/1 -> Equal8/2
  AND19/1 -> Switch34/2
  Switch14/1 -> Add6/2  "VVMC_ACCDeltaTqPGain_Nm"
  Constant58/1 -> Switch14/1
  Switch34/1 -> Switch33/3
  Constant57/1 -> Equal2/2
  [VVMC_FeatArbitrFinal_enum] -> Relational Operator17/1
  Relational Operator17/1 -> AND11/2
  MVMC_ACCDeltaTqPGain_Z_Nm1/1 -> Switch14/3
  [VVMC_FeatSetSpdForCalcu_kph] -> u2 > 0/1
  Relational Operator6/1 -> u2 > 0 (1)/2
  AND11/1 -> Switch14/2
  Equal7/1 -> AND17/2
  Constant14/1 -> Saturation Dynamic5/1
  Constant22/1 -> u2 > 0 (1)/3
  Constant123/1 -> Relational Operator55/2
  Switch81/1 -> [VVMC_ACCDeltaAccel_mps2], Saturation Dynamic4/2  "VVMC_ACCDeltaAccel_mps2"
  [VVMC_VehicleSpeed_kph] -> MVMC_ACCDeltaTqPGain_Z_Nm1/2
  Add8/1 -> Saturation Dynamic5/2
  Equal6/1 -> AND17/1
  [VVMC_VehicleSpeed_kph] -> MVMC_ACCDeltaTqIGain_Z_Nm/2
  Constant9/1 -> Product1/2
  Relational Operator55/1 -> Switch33/2
  [VVMC_FeatArbitrFinal_enum] -> Relational Operator55/1
  Constant13/1 -> Saturation Dynamic4/1
  MVMC_ACCDeltaTqIGain_Z_Nm/1 -> Switch26/3  "VVMC_ACCDeltaTqIGainOri_Nm"
  Relational Operator5/1 -> u2 > 0/2
  Data Type Conversion1/1 -> Add8/1
  Constant124/1 -> Equal6/2
  MVMC_DISCDeltaTqIGain_Z_Nm/1 -> Switch40/1, [VVMC_DISCDeltaTqIGain_Nm]  "VVMC_DISCDeltaTqIGain_Nm"
  [VINP_TargetType_enum] -> Equal2/1
  Constant125/1 -> Equal7/2
  [VVMC_VehicleSpeed_kph] -> MVMC_DISCDeltaTqIGain_Z_Nm/2
  [VVMC_ActACCRequiredAccel_mps2] -> Equal7/1
  AND17/1 -> AND19/1
  [VVMC_LongAcc_Gps] -> Equal6/1
  [VVMC_MeterIndSpeedForCalcu_kph] -> Add8/2
  u2 > 0 (1)/1 -> u2 > 0/3
  u2 > 0/1 -> Data Type Conversion1/1
  Constant60/1 -> Relational Operator17/2
  Constant21/1 -> Relational Operator6/2
  Product1/1 -> Add7/2
  Equal2/1 -> AND11/1
  Constant15/1 -> Saturation Dynamic5/3
  [VVMC_FeatReqSpd_kph] -> u2 > 0 (1)/1
  [VVMC_FeatArbitrFinal_enum] -> Relational Operator5/1
  [VVMC_FeatArbitrFinal_enum] -> Relational Operator6/1
  Constant16/1 -> Relational Operator5/2
  [VVMC_LongAcc_Gps] -> Product1/1
  Saturation Dynamic5/1 -> MVMC_ACCDeltaTqPGain_Z_Nm1/1  "VVMC_ACCActSpdDev_kph"
  Switch33/1 -> Add6/1  "VVMC_ACCDeltaTqIGain_Nm"
  Saturation Dynamic4/1 -> [VVMC_ActAccDev_mps2]  "VVMC_ActAccDev_mps2"
  Constant12/1 -> Saturation Dynamic4/3
  [VVMC_ADASNegReq_flg] -> NOT13/1
  NOT13/1 -> AND8/1
  AND8/1 -> Switch27/2
  Relational Operator49/1 -> AND14/1
  Constant59/1 -> Divide2/2
  [VVMC_ACCDeltaTq_Nm] -> Add5/2
  Divide3/1 -> Add15/2
  Constant41/1 -> Relational Operator20/2
  Constant91/1 -> Relational Operator40/2
  SR_Latch6/1 -> [VVMC_ACCLowSpdTqCtrl_flg]  "VVMC_ACCLowSpdTqCtrl_flg"
  [VTQD_CoordWhlTqDemRr_Nm] -> Add9/2
  [VVMC_ACCLowSpdTqCtrl_flg] -> Switch18/2
  Constant51/1 -> Add/1
  [VVMC_VehicleSpeed_kph] -> Add3/2
  Relational Operator33/1 -> Logical Operator5/2
  Constant116/1 -> Relational Operator50/2
  Triggered Subsystem1/1(Out1) -> [VVMC_ACCLowSpdTqLimit_Nm]  "VVMC_ACCLowSpdTqLimit_Nm"
  [VVMC_ACCLowSpdTqLimit_Nm] -> Add10/2
  [VVMC_LastADASWhlTqCal_Nm] -> Add1/1
  [VVMC_ACCDeltaTq_Nm] -> Add1/2
  Relational Operator14/1 -> Logical Operator/3
  [VVMC_ActACCRequiredAccel_mps2] -> Relational Operator14/1
  Constant42/1 -> Divide1/2
  Relational Operator40/1 -> Logical Operator8/5
  Constant45/1 -> Relational Operator15/2
  Constant66/1 -> Relational Operator23/2
  Relational Operator22/1 -> Logical Operator2/5
  Constant37/1 -> Relational Operator12/2
  Constant50/1 -> Add10/1
  Constant85/1 -> Divide5/3
  Relational Operator24/1 -> Switch17/2
  Divide5/1 -> Add13/2
  [VVMC_ADASNegReq_flg] -> Detect Decrease2/1
  Add3/1 -> Divide/1
  [VVMC_LastADASWhlTqCal_Nm] -> Add15/1
  Add4/1 -> Divide/2
  Add12/1 -> Relational Operator9/2, Switch10/3  "VVMC_ACCTqRampOutByMCP_Nm"
  Relational Operator9/1 -> Switch10/2
  Constant52/1 -> Min1/2
  AND/1 -> Logical Operator1/3
  Logical Operator5/1 -> Switch12/2
  Constant112/1 -> Relational Operator47/2
  Add10/1 -> Divide/3
  [VVMC_VehicleSpeed_kph] -> Relational Operator11/1
  Unit Delay6/1 -> Relational Operator29/1
  Relational Operator10/1 -> Logical Operator3/2
  Constant62/1 -> Relational Operator21/2
  Relational Operator21/1 -> Logical Operator2/4
  Switch27/1 -> Switch12/1  "VVMC_ACCLowSpdTqEnSpdHi_Nm"
  [VTQR_FrTMTqReq_Nm] -> Unit Delay18/1
  [VVMC_ActACCRequiredAccel_mps2] -> Relational Operator22/1
  Relational Operator23/1 -> Logical Operator2/3
  OR3/1 -> Triggered Subsystem1/Trigger, SR_Latch6/1
  [VVMC_ACCLowSpdTqCtrl_flg] -> Logical Operator5/1
  Switch22/1 -> Unit Delay7/1, [VVMC_ACCLowSpdTq_Nm]  "VVMC_ACCLowSpdTq_Nm"
  Constant38/1 -> Divide1/3
  AND14/1 -> AND13/3
  Relational Operator26/1 -> Switch19/2
  Unit Delay3/1 -> Relational Operator25/1
  [VVMC_VehicleSpeed_kph] -> Triggered Subsystem1/2(In2)
  [VVMC_VehicleSpeed_kph] -> Unit Delay/1
  Switch24/1 -> Switch23/3, Max1/1
  Relational Operator41/1 -> Logical Operator8/4
  Constant40/1 -> Relational Operator14/2
  [VVMC_ActACCRequiredAccel_mps2] -> Relational Operator28/1
  Relational Operator28/1 -> Logical Operator4/4
  [VVMC_ADASActive_flg] -> Detect Increase1/1
  Constant72/1 -> Relational Operator28/2
  Relational Operator42/1 -> Logical Operator8/3
  Constant73/1 -> Relational Operator29/2
  Logical Operator4/1 -> OR3/1
  Constant75/1 -> Relational Operator30/2
  Constant77/1 -> Relational Operator31/2
  [VVMC_ZeroRgnTqSpdCtrlTq_Nm] -> Add14/2
  [VVMC_ACCLowSpdCtrlEnSpd_kph] -> Relational Operator33/1
  [VVMC_VehicleSpeed_kph] -> Relational Operator32/1
  Constant79/1 -> Relational Operator33/2
  Constant78/1 -> Relational Operator32/2
  Detect Increase4/1 -> Switch22/2
  Max3/1 -> Switch29/1
  Unit Delay5/1 -> Add11/2
  Constant4/1 -> Relational Operator24/2
  [VVMC_ACCLowSpdTqCtrl_flg] -> Detect Increase4/1
  Constant47/1 -> Add3/1
  Relational Operator43/1 -> Logical Operator9/3
  Max/1 -> Max3/1
  Relational Operator47/1 -> AND8/2
  Relational Operator20/1 -> AND13/1
  Min1/1 -> Switch42/3
  [VVMC_ACCLowSpdCtrlEnSpd_kph] -> Add4/2
  [VVMC_ActACCRequiredAccel_mps2] -> Relational Operator24/1
  Add9/1 -> Switch8/1
  Constant117/1 -> Max3/2
  Switch15/1 -> Add12/2
  Switch12/1 -> Max/1, Switch29/3, Relational Operator50/1, Switch22/1
  [VVMC_LastACCLowSpdTq_Nm] -> Max/2
  Relational Operator12/1 -> Logical Operator/1
  Constant99/1 -> Add14/1
  Max2/1 -> Switch24/1
  Constant53/1 -> Switch21/1
  [task_time_s] -> Divide3/3
  [VVMC_VehicleSpeed_kph] -> Relational Operator31/1
  [VVMC_RgnProhibited_flg] -> Switch23/2
  Constant89/1 -> Max1/2
  Constant100/1 -> Divide3/2
  Add1/1 -> Switch8/3
  Switch18/1 -> Switch24/3
  [VVMC_ActACCRequiredAccel_mps2] -> Unit Delay9/1
  Constant6/1 -> Relational Operator8/2
  Constant98/1 -> Relational Operator45/2
  Relational Operator45/1 -> Logical Operator8/2
  Relational Operator29/1 -> Logical Operator4/3
  Add/1 -> Max4/2
  [VVMC_ADASActive_flg] -> NOT9/1
  Constant97/1 -> Relational Operator44/2
  [VVMC_ActACCRequiredAccel_mps2] -> Relational Operator43/1
  [VVMC_ActACCRequiredAccel_mps2] -> Unit Delay6/1
  Switch21/1 -> Switch12/3  "VVMC_ACCLowSpdTqEnSpdLo_Nm"
  Relational Operator30/1 -> Logical Operator4/2
  Relational Operator44/1 -> Logical Operator9/1
  Constant67/1 -> Relational Operator25/2
  Divide/1 -> Add/2
  [VVMC_VehicleSpeed_kph] -> Relational Operator40/1
  Constant96/1 -> Relational Operator43/2
  [VVMC_LastADASWhlTqCal_Nm] -> Triggered Subsystem4/1(In1)
  Relational Operator32/1 -> Logical Operator2/1, Logical Operator4/5
  [VVMC_LastADASWhlTqCal_Nm] -> Relational Operator45/1
  Add13/1 -> Add23/1, Switch36/3
  Detect Decrease2/1 -> Switch8/2
  Unit Delay9/1 -> Relational Operator42/1
  Triggered Subsystem4/1(Out1) -> [VVMC_ZeroRgnTqSpdCtrlTq_Nm]  "VVMC_ZeroRgnTqSpdCtrlTq_Nm"
  Divide1/1 -> Add13/1
  Add5/1 -> Switch6/1
  Add15/1 -> Max2/1  "VVMC_ADASWhlTqCalZeroRgnCtrl_Nm"
  [VVMC_ZeroRgnTqSpdCtrl_flg] -> Switch24/2
  Detect Increase1/1 -> AND32/1
  Unit Delay7/1 -> [VVMC_LastACCLowSpdTq_Nm]
  Add11/1 -> Divide2/1
  Saturation Dynamic7/1 -> [VVMC_OriADASWhlTq_Nm]  "VVMC_OriADASWhlTq_Nm"
  Logical Operator8/1 -> Triggered Subsystem4/Trigger, SR_Latch4/1
  Switch6/1 -> Cast To Single2/1
  NOT9/1 -> Logical Operator9/4
  Triggered Subsystem1/2(Out2) -> [VVMC_ACCLowSpdCtrlEnSpd_kph]  "VVMC_ACCLowSpdCtrlEnSpd_kph"
  [VTQR_RrTMTqReq_Nm] -> Unit Delay19/1
  Min2/1 -> Switch16/3  "VVMC_ACCTqNegReq_Nm"
  Constant64/1 -> Relational Operator22/2
  Switch10/1 -> Min2/1
  [VVMC_VehicleSpeed_kph] -> Relational Operator44/1
  [VVMC_MCPresBaseTq_Nm] -> Add1/4
  Constant70/1 -> Relational Operator26/2
  Switch23/1 -> Switch17/3  "VVMC_ADASWhlTqCalNegCMD_Nm"
  Constant101/1 -> Max2/2
  Add14/1 -> Divide3/1
  Constant69/1 -> Switch15/3
  AND13/1 -> Switch21/2
  Constant114/1 -> Relational Operator49/2
  [VVMC_ActACCRequiredAccel_mps2] -> Relational Operator10/1
  Relational Operator15/1 -> Logical Operator/4
  Constant84/1 -> Divide5/2
  Constant92/1 -> Relational Operator41/2
  Divide2/1 -> Switch15/2, Switch15/1
  [VTQD_CoordWhlTqDemFr_Nm] -> Add9/1
  [VINP_MCPressure_bar] -> Unit Delay5/1, Add11/1
  NOT1/1 -> Logical Operator3/3
  Constant36/1 -> Relational Operator11/2
  Logical Operator1/1 -> Switch6/2
  [VVMC_TMSpdBaseTq_Nm] -> Add1/3
  Unit Delay/1 -> Relational Operator12/1
  Relational Operator8/1 -> Logical Operator3/1
  Constant29/1 -> Relational Operator10/2
  Logical Operator3/1 -> SR_Latch6/2
  Constant63/1 -> Min2/2
  [VVMC_ADASActive_flg] -> NOT1/1
  [VVMC_VehicleSpeed_kph] -> Relational Operator8/1
  [VVMC_LastADASWhlTqCal_Nm] -> Add12/1
  Logical Operator/1 -> OR3/3
  Max1/1 -> Switch23/1
  Relational Operator25/1 -> Logical Operator2/2
  Constant93/1 -> Relational Operator42/2
  Logical Operator2/1 -> OR3/2
  [VVMC_ActACCRequiredAccel_mps2] -> Relational Operator41/1
  Relational Operator31/1 -> Logical Operator4/1
  Constant48/1 -> Add4/1
  SR_Latch4/1 -> [VVMC_ZeroRgnTqSpdCtrl_flg]  "VVMC_ZeroRgnTqSpdCtrl_flg"
  Relational Operator11/1 -> Logical Operator/2
  [VVMC_VehicleSpeed_kph] -> Relational Operator20/1
  [VVMC_VehicleSpeed_kph] -> Relational Operator21/1
  Switch29/1 -> Switch22/3
  Constant119/1 -> Switch/1
  NOT2/1 -> AND2/1
  Min/1 -> MVMC_TMSpdBaseTq_Y_Nm/1
  Equal1/1 -> AND10/1
  [VVMC_EstSlope_Deg] -> Equal3/1
  Constant55/1 -> Equal3/2
  AND10/1 -> Switch13/2
  [VINP_MCPressure_bar] -> Relay1/1
  Constant54/1 -> Equal1/2
  Switch/1 -> [VVMC_TMSpdBaseTq_Nm]  "VVMC_TMSpdBaseTq_Nm"
  Relay1/1 -> Switch13/3
  Equal3/1 -> AND10/2
  [VVMC_VehicleSpeed_kph] -> Equal1/1
  [VINP_MCPressure_bar] -> Relay/1
  Constant110/1 -> Equal5/2
  [VINP_FrTMSpd_rpm] -> Min/1
  [VVMC_VehicleSpeed_kph] -> Equal5/1
  Equal5/1 -> AND2/3
  [VVMC_MCPreBaseTqEn_flg] -> NOT2/1
  [VINP_RrTMSpd_rpm] -> Min/2
  AND2/1 -> [VVMC_ADASNegReq_flg]  "VVMC_ADASNegReq_flg"
  Switch13/1 -> AND2/2  "VVMC_ADASNegReqAct_flg"
  Relay/1 -> Switch13/1
  [VVMC_ACCVehHoldReqRaw_flg] -> Switch/2
  MVMC_TMSpdBaseTq_Y_Nm/1 -> Switch/3
  task_time_s/1 -> [task_time_s]
  [VVMC_ACCLowSpdTqCtrl_flg] -> VVMC_ACCLowSpdTqCtrl_flg/1
  VTQR_FrTMTqReq_Nm/1 -> [VTQR_FrTMTqReq_Nm]
  VVMC_SafetyCtrl_flg/1 -> [VVMC_SafetyCtrl_flg]
  VINP_TargetType_enum/1 -> [VINP_TargetType_enum]
  VVMC_EstSlope_Deg/1 -> [VVMC_EstSlope_Deg]
  Constant56/1 -> Relational Operator16/2
  Relational Operator16/1 -> AND3/3
  [VVMC_EstSlope_Deg] -> Relational Operator16/1
  VVMC_ACCVehHoldReqRaw_flg/1 -> [VVMC_ACCVehHoldReqRaw_flg]
  VTQR_RrTMTqReq_Nm/1 -> [VTQR_RrTMTqReq_Nm]
  [VVMC_ADASNegReq_flg] -> VVMC_ADASNegReq_flg/1
  Constant5/1 -> Switch3/2
  Switch3/1 -> [VVMC_FrntAxlTrqReqBrk_Nm]  "VVMC_FrntAxlTrqReqBrk_Nm"
  Switch4/1 -> [VVMC_RearAxlTrqReqBrk_Nm]  "VVMC_RearAxlTrqReqBrk_Nm"
  Constant26/1 -> Switch4/2
  Constant27/1 -> Switch4/3
  Constant25/1 -> Switch3/3
  [VINP_RearAxlTrqReqBrk_Nm] -> Switch4/1
  [VINP_FrntAxlTrqReqBrk_Nm] -> Switch3/1
  [VVMC_SWCResUpSta_flg] -> Detect Increase3/1
  Constant31/1 -> Relational Operator7/2
  [VVMC_ActACCRequiredAccel_mps2] -> Relational Operator7/1
  AND4/1 -> SR_Latch/1
  [VVMC_SWCResUpSta_flg] -> Detect Increase2/1
  VVMC_MeterIndSpeedForCalcu_kph/1 -> [VVMC_MeterIndSpeedForCalcu_kph]
  VTQD_SWC2ResUpSta_flg/1 -> [VTQD_SWC2ResUpSta_flg]
  VINP_FrntAxlTrqReqBrk_Nm/1 -> [VINP_FrntAxlTrqReqBrk_Nm]
  VINP_RearAxlTrqReqBrk_Nm/1 -> [VINP_RearAxlTrqReqBrk_Nm]
  VVMC_FeatSetSpdForCalcu_kph/1 -> [VVMC_FeatSetSpdForCalcu_kph]
  VVMC_ACCPedalOvrd_flg/1 -> [VVMC_ACCPedalOvrd_flg]
  VTQD_CoordWhlTqDemRr_Nm/1 -> [VTQD_CoordWhlTqDemRr_Nm]
  VTQD_CoordWhlTqDemFr_Nm/1 -> [VTQD_CoordWhlTqDemFr_Nm]
  [VVMC_ADASWhlTqCal_Nm] -> VVMC_ADASWhlTqCal_Nm/1
  VVMC_ADASActive_flg/1 -> [VVMC_ADASActive_flg]
  VVMC_VehicleSpeed_kph/1 -> [VVMC_VehicleSpeed_kph]
  VVMC_ActACCRequiredAccel_mps2/1 -> [VVMC_ActACCRequiredAccel_mps2]
  VVMC_LongAcc_Gps/1 -> [VVMC_LongAcc_Gps]
  VVMC_FeatArbitrFinal_enum/1 -> [VVMC_FeatArbitrFinal_enum]
  VINP_ESCADASSta_enum/1 -> [VINP_ESCADASSta_enum]
  VINP_MCPressure_bar/1 -> [VINP_MCPressure_bar]
  VINP_RrTMSpd_rpm/1 -> [VINP_RrTMSpd_rpm]
  VINP_FrTMSpd_rpm/1 -> [VINP_FrTMSpd_rpm]
  Relational Operator3/1 -> OR1/1
  Constant20/1 -> Relational Operator/2
  Constant3/1 -> Equal/2
  SR_Latch1/1 -> AND3/4  "VVMC_HillUpESCStaEn_flg"
  AND3/1 -> [VVMC_MCPreBaseTqEn_flg]  "VVMC_MCPreBaseTqEn_flg"
  SR_Latch/1 -> AND3/1  "VVMC_HillUpHoldReqEn_flg"
  Detect Increase3/1 -> AND1/2
  Constant2/1 -> Relational Operator2/2
  Constant7/1 -> Relational Operator4/2
  [VINP_FrTMSpd_rpm] -> Relational Operator3/1
  [VVMC_MCPreBaseTqEn_flg] -> Switch1/2
  Relational Operator4/1 -> OR1/2
  Constant8/1 -> Relational Operator3/2
  Constant19/1 -> Switch1/3
  OR1/1 -> SR_Latch1/2
  Relational Operator2/1 -> OR/2
  AND1/1 -> SR_Latch1/1
  [VINP_RrTMSpd_rpm] -> Relational Operator4/1
  [VINP_ESCADASSta_enum] -> Equal/1
  [VINP_FrTMSpd_rpm] -> Relational Operator/1
  OR/1 -> SR_Latch/2
  Equal/1 -> AND1/1
  Relational Operator/1 -> OR/1
  [VINP_MCPressure_bar] -> Switch1/1
  Switch1/1 -> MVMC_MCPresBaseTq_Y_Nm/1
  MVMC_MCPresBaseTq_Y_Nm/1 -> [VVMC_MCPresBaseTq_Nm]  "VVMC_MCPresBaseTq_Nm"
  [VVMC_ACCVehHoldReqRaw_flg] -> AND4/1
  [VINP_RrTMSpd_rpm] -> Relational Operator2/1
  VVMC_FeatReqSpd_kph/1 -> [VVMC_FeatReqSpd_kph]
  VVMC_ReqBrkJoin_flg/1 -> [VVMC_ReqBrkJoin_flg]
  AND15/1 -> Switch40/2
  NOT11/1 -> AND15/2
  [VVMC_ReqBrkJoin_flg] -> Unit Delay14/1
  Unit Delay14/1 -> NOT11/1
  Switch71/1 -> MVMC_VehHoldTqIncGain_Y_Nm/1, 1-D Lookup Table/1
  1-D Lookup Table/1 -> [VVMC_ACCDeltaTqGradeGn_Nm]  "VVMC_ACCDeltaTqGradeGn_Nm"
  [VVMC_ACCDeltaTq_Nm] -> Add9/3
  [VVMC_RearAxlTrqReqBrk_Nm] -> Add26/2
  Constant39/1 -> AND21/1
  [VVMC_FrntAxlTrqReqBrk_Nm] -> Add26/1
  Unit Delay16/1 -> Add27/2
  Add27/1 -> Switch38/1
  Add26/1 -> Unit Delay16/1, Add27/1
  Constant46/1 -> Switch38/3
  Switch38/1 -> [VVMC_ADSBRgnDeltaTq_Nm]  "VVMC_ADSBRgnDeltaTq_Nm"
  [VVMC_ADSBRgnDeltaTq_Nm] -> Add20/2
  [VVMC_OriADASWhlTq_Nm] -> Relational Operator15/1, Relational Operator30/1, Unit Delay3/1, Relational Operator23/1
  [VVMC_OriADASWhlTq_Nm] -> Relational Operator49/1
  [VVMC_OriADASWhlTq_Nm] -> Switch21/3
  [VVMC_OriADASWhlTq_Nm] -> Switch19/1
  [VVMC_OriADASWhlTq_Nm] -> Relational Operator26/1
  [VVMC_OriADASWhlTq_Nm] -> Switch16/1
  [VVMC_OriADASWhlTq_Nm] -> Switch10/1, Relational Operator9/1
  [VVMC_ACCLowSpdTq_Nm] -> Switch20/3
  Switch17/1 -> [VVMC_ADASWhlTqCalBftHold_Nm]  "VVMC_ADASWhlTqCalBftHold_Nm"
  [VVMC_ADASWhlTqCalBftHold_Nm] -> Switch11/1
  [VVMC_ADASWhlTqCalBftHold_Nm] -> Switch30/1
  [VVMC_ADASWhlTqCalBftHold_Nm] -> Relational Operator51/1
  [VVMC_OriADASWhlTq_Nm] -> Switch17/1
  [VVMC_ADASWhlTqCalAftHold_Nm] -> u2 > 0 (3)/3
  Constant1/1 -> Switch42/2
  Switch42/1 -> Switch27/3
  [VVMC_OriADASWhlTq_Nm] -> Relational Operator47/1
  Constant49/1 -> Logical Operator7/2
  Constant76/1 -> Logical Operator9/2
  Constant113/1 -> NOT12/1
  AND16/1 -> Switch29/2
  NOT12/1 -> AND16/2
  [VVMC_ActAccDev_mps2] -> MVMC_DISCDeltaTqIGain_Z_Nm/1
  [VVMC_ActAccDev_mps2] -> MVMC_ACCDeltaTqIGain4OVRD_Z_Nm/1
  [VVMC_ActAccDev_mps2] -> MVMC_ACCDeltaTqIGain_Z_Nm/1
  [VVMC_OriADASWhlTq_Nm] -> Switch27/1
  [VVMC_OriADASWhlTq_Nm] -> Max4/1
  Constant156/1 -> Max12/2
  Equal13/1 -> AND7/2
  AND7/1 -> Switch28/2
  [VVMC_EstSlope_Deg] -> Equal13/1
  Constant28/1 -> Equal13/2
  Constant32/1 -> Switch25/2
  Switch25/1 -> [VVMC_VehHoldCtrlTq_Nm]
  Saturation Dynamic2/1 -> [VVMC_ADASWhlTqCalVehHoldPosTq_Nm], Switch28/3  "VVMC_ADASWhlTqCalVehHoldPosTq_Nm"
  Add20/1 -> Switch42/1  "VVMC_ACCRgnTq2Hold_Nm"
  [VVMC_LongAcc_Gps] -> Equal14/1
  Constant130/1 -> Equal14/2
  Equal14/1 -> AND29/1
  [VVMC_ACCDeltaTqGradeGn_Nm] -> Max10/1
  [VVMC_ACCDeltaTqGradeGn_Nm] -> Switch25/3
  [VVMC_ADASWhlTqCalBftHold_Nm] -> Max12/1
  Max12/1 -> Switch39/1
  Constant134/1 -> NOT14/1
  NOT14/1 -> AND13/2
  ic0/1 -> [VVMC_LastADASWhlTqCal_Nm]  "VVMC_LastADASWhlTqCal_Nm"
  Switch49/1 -> [VVMC_ACCDeltaTq_Nm]  "VVMC_ACCDeltaTq_Nm"
  [VVMC_ADASNegReq_flg] -> Switch49/2
  Switch2/1 -> [VVMC_SWCResUpSta_flg]
  Constant135/1 -> Divide9/1
  [VVMC_ACCWhlTqLowerLim_Nm] -> VVMC_ACCWhlTqLowerLim_Nm/1
  MVMC_VehHoldTqIncGain_Y_Nm/1 -> [VVMC_UphillTqIncSR_Nm]
  [VVMC_UphillTqIncSR_Nm] -> Switch31/1
  [VTQD_CreepBaseTqD_Nm] -> Max10/2
  Max10/1 -> Switch25/1
  Add6/1 -> Switch49/3, Switch32/3, Switch44/2, Divide9/2
  Divide9/1 -> Switch44/3
  Switch44/1 -> Switch49/1
  Constant34/1 -> Saturation Dynamic6/1
  [VVMC_OriADASWhlTq_Nm] -> Saturation Dynamic6/2
  MVMC_ACCLoSpdTqLowerLim_Z_Nm/1 -> Saturation Dynamic6/3
  [VVMC_VehicleSpeed_kph] -> MVMC_ACCLoSpdTqLowerLim_Z_Nm/2
  Switch52/1 -> MVMC_ACCLoSpdTqLowerLim_Z_Nm/1, Unit Delay28/1
  [VVMC_LastADASWhlTqCal_Nm] -> Switch35/2
  Switch35/1 -> Switch56/1
  Max8/1 -> Switch35/1
  [VVMC_LastADASWhlTqCal_Nm] -> Add16/1
  Divide7/1 -> Add16/2, Add21/2
  Add16/1 -> Max5/1
  Constant43/1 -> Max5/2
  Max5/1 -> Switch35/3
  AND21/1 -> Switch38/2
  [VVMC_ACCLowSpdTqCtrl_flg] -> Unit Delay12/1
  Unit Delay12/1 -> AND21/2
  [VINP_RrTMSpd_rpm] -> MVMC_TMRevPrvtTq_Y_Nm/1, Relational Operator57/1
  Constant65/1 -> Relational Operator57/2
  Relational Operator57/1 -> SR_Latch7/1
  Constant83/1 -> Switch43/3
  Constant95/1 -> Relational Operator59/2
  [VINP_RrTMSpd_rpm] -> Relational Operator59/1
  Relational Operator59/1 -> SR_Latch7/2
  SR_Latch7/1 -> Switch43/2, [VVMC_TMRevPrvtEn_flg]
  MVMC_TMRevPrvtTq_Y_Nm/1 -> Switch43/1
  Switch43/1 -> [VVMC_TMRevPrvtTq_Nm]  "VVMC_TMRevPrvtTq_Nm"
  [VVMC_TMRevPrvtTq_Nm] -> Add22/2
  Max9/1 -> Saturation Dynamic2/2
  [VVMC_TMRevPrvtTq_Nm] -> Add17/3
  Add25/1 -> Max9/1
  Constant102/1 -> Switch45/3
  Constant105/1 -> Switch45/2
  [VVMC_ADASWhlTqCalVehHoldPosTq_Nm] -> Switch45/1
  Saturation Dynamic6/1 -> Add20/1
  [VVMC_UphillTqIncSRFinal_Nm] -> Add22/1
  Switch32/1 -> Switch44/1
  Constant35/1 -> Switch32/2
  Constant111/1 -> Switch32/1
  Constant115/1 -> AND22/2
  [VVMC_TMRevPrvtEn_flg] -> AND22/1
  AND22/1 -> Switch46/2
  [VVMC_TMRevPrvtTq_Nm] -> Add18/2
  Unit Delay15/1 -> Add18/1
  Add18/1 -> Switch46/1
  Switch46/1 -> Unit Delay15/1, Add25/1
  [VVMC_TMRevPrvtTq_Nm] -> Switch46/3
  Constant118/1 -> AND5/2
  Relational Operator107/1 -> AND23/1
  Constant121/1 -> AND23/2
  AND23/1 -> Switch47/2
  Max6/1 -> Switch47/3
  Constant126/1 -> Switch47/1
  Constant127/1 -> Switch48/2
  Switch48/1 -> Switch41/3  "VVMC_ADASWhlTqVehHoldBfrSS_Nm"
  [VVMC_VHJerkPrvtTq_Nm] -> Switch48/1
  Constant128/1 -> Relational Operator60/2
  [VVMC_VehicleSpeed_kph] -> Relational Operator60/1
  Relational Operator60/1 -> Switch50/2
  Switch50/1 -> [VVMC_VHJerkPrvtTq_Nm]  "VVMC_VHJerkPrvtTq_Nm"
  [VVMC_TMRevPrvtTq4JertPrvt_Nm] -> Add24/2
  [VVMC_LastADASWhlTqCal_Nm] -> Add24/1
  Add24/1 -> Switch50/3
  [VINP_RrTMSpd_rpm] -> MVMC_TMRevPrvtTq4JP_Z_Nm/2
  Switch51/1 -> [VVMC_TMRevPrvtTq4JertPrvt_Nm]  "VVMC_TMRevPrvtTq4JertPrvt_Nm"
  Unit Delay18/1 -> Divide1/1
  Unit Delay19/1 -> Divide5/1
  Min3/1 -> u2 > 0 (4)/1
  [VVMC_ADASWhlTqCalAftHold_Nm] -> Min3/2
  [VVMC_LastADASWhlTqCal_Nm] -> Min3/1
  [VVMC_LastADASWhlTqCal_Nm] -> Min4/1
  [VVMC_ADASWhlTqCalAftHold_Nm] -> Min4/2
  Min4/1 -> u2 > 0 (4)/3
  Constant145/1 -> Relational Operator18/2
  [VINP_RDCActive_enum] -> Relational Operator18/1
  Relational Operator18/1 -> OR5/4
  VINP_RDCActive_enum/1 -> [VINP_RDCActive_enum]
  [VINP_RDCActive_enum] -> Detect Change1/1
  Detect Change1/1 -> AND24/1
  [VINP_RDCActive_enum] -> Relational Operator64/1
  Constant147/1 -> Relational Operator64/2
  Relational Operator64/1 -> AND24/2
  AND24/1 -> Logical Operator1/1
  Switch53/1 -> Unit Delay26/1, MVMC_ACCLoSpdTqLoLim4JP_Z_Nm/1
  [VVMC_VehicleSpeed_kph] -> MVMC_ACCLoSpdTqLoLim4JP_Z_Nm/2
  Cast To Single2/1 -> Saturation Dynamic7/2
  Constant146/1 -> Saturation Dynamic7/1
  MVMC_ACCLoSpdTqLoLim4JP_Z_Nm/1 -> Saturation Dynamic7/3
  Unit Delay25/1 -> Switch53/2
  [VVMC_EstSlope_Deg] -> Switch53/3
  [VVMC_VehicleSpeed_kph] -> Relational Operator65/1
  Constant149/1 -> Relational Operator65/2
  Relational Operator65/1 -> AND25/2
  [VVMC_ACCVehHoldReqRaw_flg] -> AND25/1
  AND25/1 -> SR_Latch9/1
  NOT10/1 -> SR_Latch9/2
  [VVMC_ACCVehHoldReqRaw_flg] -> NOT10/1
  [VINP_RrTMSpd_rpm] -> Triggered Subsystem/1(In1)
  SR_Latch9/1 -> [VVMC_VHZeroVehSpd_flg], Triggered Subsystem/Trigger
  Triggered Subsystem/1(Out1) -> [VVMC_ZeroSpdEnTMSpd_rpm]  "VVMC_ZeroSpdEnTMSpd_rpm"
  Constant150/1 -> Divide8/1
  [task_time_s] -> Divide8/2
  Divide8/1 -> Add29/2
  Switch54/1 -> Add29/1
  Constant151/1 -> Max7/2
  Add29/1 -> Max7/1
  Max7/1 -> [VVMC_ZeroSpdTMSpdCtrlTarget_rpm]  "VVMC_ZeroSpdTMSpdCtrlTarget_rpm"
  [VVMC_ZeroSpdTMSpdCtrlTarget_rpm] -> Add30/1
  [VINP_RrTMSpd_rpm] -> Add30/2
  Add30/1 -> MVMC_VHTMSpdCtrl_Z_Nm/2
  Switch60/1 -> [VVMC_VHTMSpdCtrlDeltaTq_Nm]  "VVMC_VHTMSpdCtrlDeltaTq_Nm"
  [VVMC_VHTMSpdCtrlDeltaTq_Nm] -> Add24/3
  Detect Increase/1 -> Switch54/2
  [VVMC_VHZeroVehSpd_flg] -> Detect Increase/1
  [VVMC_ZeroSpdEnTMSpd_rpm] -> Switch54/1
  [VVMC_ZeroSpdTMSpdCtrlTarget_rpm] -> Unit Delay20/1
  Unit Delay20/1 -> Switch54/3
  Saturation Dynamic3/1 -> [VVMC_ADASWhlTqCalBftZC_Nm]  "VVMC_ADASWhlTqCalBftZC_Nm"
  [VVMC_LastADASWhlTqCal_Nm] -> Relational Operator66/1
  Constant144/1 -> Relational Operator66/2
  [VVMC_ADASWhlTqCalBftZC_Nm] -> Relational Operator67/1
  Constant137/1 -> Relational Operator67/2
  Relational Operator67/1 -> AND26/2
  Relational Operator66/1 -> AND26/1
  AND31/1 -> Switch55/2
  [VVMC_ADASWhlTqCalBftZC_Nm] -> Switch55/3
  AND26/1 -> Triggered Subsystem2/Trigger, SR_Latch10/1
  SR_Latch10/1 -> [VVMC_ZCNegDetEn_flg]  "VVMC_ZCNegDetEn_flg"
  Relational Operator68/1 -> OR2/1
  [VVMC_ADASWhlTqCalBftZC_Nm] -> Relational Operator80/1
  [VVMC_NegZCHoldTq_Nm] -> Relational Operator80/2
  Relational Operator80/1 -> OR10/2
  Relational Operator79/1 -> OR10/1
  OR10/1 -> SR_Latch12/2
  AND40/1 -> Timer2/1, NOT17/1
  NOT17/1 -> Timer2/2
  [VVMC_ZCWaitTimeNeg_s] -> Relational Operator79/2, Timer2/4
  Timer2/1 -> Relational Operator79/1
  [task_time_s] -> Timer2/3
  SR_Latch12/1 -> [VVMC_ZCNegCtrlEn_flg]  "VVMC_ZCNegCtrlEn_flg"
  AND28/1 -> SR_Latch12/1
  Relational Operator76/1 -> AND28/2
  Relational Operator77/1 -> AND28/3
  [VVMC_NegZCHoldTq_Nm] -> Relational Operator77/2
  [VVMC_ADASWhlTqCalBftZC_Nm] -> Relational Operator77/1
  [VVMC_NegZCHoldTq_Nm] -> Relational Operator76/2
  [VVMC_LastADASWhlTqCal_Nm] -> Relational Operator76/1
  Constant141/1 -> Relational Operator68/2
  [VVMC_ADASWhlTqCalBftZC_Nm] -> Relational Operator68/1
  Timer3/1 -> Relational Operator70/1
  [VVMC_ZCWaitTimeNeg_s] -> Relational Operator70/2, Timer3/4
  NOT15/1 -> Timer3/2
  AND37/1 -> Timer3/1, NOT15/1
  [task_time_s] -> Timer3/3
  [VVMC_ZCNegDetEn_flg] -> Unit Delay21/1
  Relational Operator70/1 -> OR2/2
  OR2/1 -> SR_Latch10/2
  [VVMC_ZCNegDetEn_flg] -> Unit Delay29/1
  [VVMC_ZCPosDetEn_flg] -> Unit Delay17/1
  OR11/1 -> SR_Latch11/2
  Relational Operator75/1 -> OR11/2
  [task_time_s] -> Timer4/3
  AND43/1 -> NOT16/1, Timer4/1
  NOT16/1 -> Timer4/2
  [VVMC_ZCWaitTimePos_s] -> Timer4/4, Relational Operator75/2
  Timer4/1 -> Relational Operator75/1
  [VVMC_ADASWhlTqCalBftZC_Nm] -> Relational Operator74/1
  Constant143/1 -> Relational Operator74/2
  [VVMC_LastADASWhlTqCal_Nm] -> Relational Operator81/1
  [VVMC_PosZCHoldTq_Nm] -> Relational Operator81/2
  [VVMC_ADASWhlTqCalBftZC_Nm] -> Relational Operator82/1
  [VVMC_PosZCHoldTq_Nm] -> Relational Operator82/2
  Relational Operator82/1 -> AND30/3
  Relational Operator81/1 -> AND30/2
  AND30/1 -> SR_Latch13/1
  SR_Latch13/1 -> [VVMC_ZCPosCtrlEn_flg]  "VVMC_ZCPosCtrlEn_flg"
  [task_time_s] -> Timer1/3
  Timer1/1 -> Relational Operator83/1
  [VVMC_ZCWaitTimePos_s] -> Timer1/4, Relational Operator83/2
  NOT18/1 -> Timer1/2
  AND46/1 -> Timer1/1, NOT18/1
  OR9/1 -> SR_Latch13/2
  Relational Operator83/1 -> OR9/1
  Relational Operator84/1 -> OR9/2
  [VVMC_PosZCHoldTq_Nm] -> Relational Operator84/2
  [VVMC_ADASWhlTqCalBftZC_Nm] -> Relational Operator84/1
  Relational Operator74/1 -> OR11/1
  SR_Latch11/1 -> [VVMC_ZCPosDetEn_flg]  "VVMC_ZCPosDetEn_flg"
  AND27/1 -> Triggered Subsystem3/Trigger, SR_Latch11/1
  Relational Operator71/1 -> AND27/1
  Relational Operator72/1 -> AND27/2
  Constant142/1 -> Relational Operator72/2
  [VVMC_ADASWhlTqCalBftZC_Nm] -> Relational Operator72/1
  Constant152/1 -> Relational Operator71/2
  [VVMC_LastADASWhlTqCal_Nm] -> Relational Operator71/1
  [VVMC_ZCNegCtrlEn_flg] -> OR12/1
  [VVMC_ZCPosCtrlEn_flg] -> OR12/2
  OR12/1 -> AND31/2
  Constant153/1 -> AND31/1
  [VINP_BrkSwSta_flg] -> NOT19/1  "VINP_BrkSwSta_flg"
  AND32/1 -> Logical Operator1/2
  NOT19/1 -> AND32/2
  VINP_BrkSwSta_flg/1 -> [VINP_BrkSwSta_flg]
  [VVMC_ACCLowSpdTqCtrl_flg] -> Unit Delay25/1
  Min6/1 -> Switch53/1
  [VVMC_EstSlope_Deg] -> Min6/2
  Unit Delay26/1 -> Min6/1
  Unit Delay28/1 -> Min7/1
  [VVMC_EstSlope_Deg] -> Min7/2
  Min7/1 -> Switch52/1
  [VVMC_ACCLowSpdTqCtrl_flg] -> Unit Delay27/1
  Unit Delay27/1 -> Switch52/2
  [VVMC_EstSlope_Deg] -> Switch52/3
  Switch56/1 -> Switch41/1
  Constant164/1 -> Relational Operator78/2
  [VINP_MCPressure_bar] -> Relational Operator78/1
  Relational Operator78/1 -> Switch56/2
  [VVMC_LastADASWhlTqCal_Nm] -> Switch56/3
  [VVMC_ZCNegCtrlEn_flg] -> Switch58/2
  Switch58/1 -> Switch55/1
  [VVMC_NegZCHoldTq_Nm] -> Switch58/1
  [VVMC_PosZCHoldTq_Nm] -> Switch58/3
  Triggered Subsystem2/1(Out1) -> MVMC_NegZCHoldTq_Y_Nm/1, MVMC_ZCWaitTimeNeg_Y_s/1
  [VVMC_VehicleSpeed_kph] -> Triggered Subsystem2/1(In1)
  MVMC_ZCWaitTimeNeg_Y_s/1 -> [VVMC_ZCWaitTimeNeg_s]  "VVMC_ZCWaitTimeNeg_s"
  MVMC_ZCWaitTimePos_Y_s/1 -> [VVMC_ZCWaitTimePos_s]  "VVMC_ZCWaitTimePos_s"
  [VVMC_VehicleSpeed_kph] -> Triggered Subsystem3/1
  Triggered Subsystem3/1 -> MVMC_PosZCHoldTq_Y_Nm/1, MVMC_ZCWaitTimePos_Y_s/1
  Unit Delay17/1 -> AND30/1
  Unit Delay29/1 -> AND28/1
  AND34/1 -> Switch60/2
  Switch75/1 -> Switch60/1
  Constant154/1 -> Switch60/3
  VINP_LFWhlRotDir_enum/1 -> [VINP_LFWhlRotDir_enum]
  VINP_LRWhlRotDir_enum/1 -> [VINP_LRWhlRotDir_enum]
  VINP_RFWhlRotDir_enum/1 -> [VINP_RFWhlRotDir_enum]
  VINP_RRWhlRotDir_enum/1 -> [VINP_RRWhlRotDir_enum]
  [VINP_RRWhlRotDir_enum] -> Relational Operator89/1
  [VINP_LRWhlRotDir_enum] -> Relational Operator88/1
  Constant173/1 -> Relational Operator88/2
  Constant174/1 -> Relational Operator89/2
  Relational Operator89/1 -> OR13/3
  Relational Operator88/1 -> OR13/1
  OR13/1 -> Switch62/2
  [VVMC_WhlDir_enum] -> MVMC_VHTMSpdCtrl_Z_Nm/1
  [VVMC_ZeroSpdTMSpdCtrlTarget_rpm] -> Relational Operator63/1
  MVMC_TMRevPrvtTq4JP_Z_Nm/1 -> Switch51/3
  Constant129/1 -> Switch51/1
  Relational Operator62/1 -> AND34/1
  [VVMC_ACCVehHoldReqRaw_flg] -> AND34/2
  Constant133/1 -> Relational Operator62/2
  [VVMC_ZeroSpdTMSpdCtrlTarget_rpm] -> Relational Operator62/1
  Constant136/1 -> Relational Operator63/2
  Relational Operator63/1 -> AND35/1
  [VVMC_ACCVehHoldReqRaw_flg] -> NOT20/1
  AND35/1 -> Switch51/2
  NOT20/1 -> AND35/2
  Constant176/1 -> Switch62/1
  Relational Operator92/1 -> OR14/1
  Relational Operator93/1 -> OR14/2
  Constant180/1 -> Relational Operator93/2
  Constant179/1 -> Relational Operator92/2
  [VINP_LRWhlRotDir_enum] -> Relational Operator92/1
  [VINP_RRWhlRotDir_enum] -> Relational Operator93/1
  OR14/1 -> OR16/1
  Switch63/1 -> Switch62/3
  Constant182/1 -> Switch63/1
  Constant181/1 -> Switch63/3
  Switch62/1 -> Cast To Single/1
  Cast To Single/1 -> [VVMC_WhlDir_enum]
  Cast To Single1/1 -> [VVMC_WhlDir4JP_enum]
  [VVMC_WhlDir4JP_enum] -> MVMC_TMRevPrvtTq4JP_Z_Nm/1
  MVMC_NegZCHoldTq_Y_Nm/1 -> [VVMC_NegZCHoldTq_Nm]  "VVMC_NegZCHoldTq_Nm"
  MVMC_PosZCHoldTq_Y_Nm/1 -> [VVMC_PosZCHoldTq_Nm]  "VVMC_PosZCHoldTq_Nm"
  VINP_FrEDURealTMTq_Nm/1 -> [VINP_FrEDURealTMTq_Nm]
  VINP_FrEDURotateDirction_enum/1 -> [VINP_FrEDURotateDirction_enum]
  VINP_RrEDURealTMTq_Nm/1 -> [VINP_RrEDURealTMTq_Nm]
  VINP_RrEDURotateDirction_enum/1 -> [VINP_RrEDURotateDirction_enum]
  [VINP_RrEDURealTMTq_Nm] -> Divide10/1
  [VINP_FrEDURealTMTq_Nm] -> Divide6/1
  Constant157/1 -> Divide6/2
  Constant158/1 -> Divide10/2
  Divide6/1 -> Add28/1
  Divide10/1 -> Add28/2
  Add28/1 -> [VVMC_TotalRealWhlTq_Nm]
  [VVMC_TotalRealWhlTq_Nm] -> Relational Operator98/1
  Constant159/1 -> Relational Operator98/2
  Relational Operator98/1 -> AND36/2
  Constant161/1 -> AND36/1
  Unit Delay21/1 -> AND36/3, AND38/1
  AND36/1 -> AND37/1
  Constant162/1 -> NOT21/1
  NOT21/1 -> AND38/2
  AND38/1 -> AND37/2
  AND41/1 -> AND40/2
  AND39/1 -> AND40/1
  NOT22/1 -> AND41/2
  [VVMC_TotalRealWhlTq_Nm] -> Relational Operator99/1
  Constant172/1 -> NOT22/1
  Relational Operator99/1 -> AND39/2
  Constant171/1 -> AND39/1
  Unit Delay23/1 -> AND39/3, AND41/1
  Constant163/1 -> Relational Operator99/2
  [VVMC_ZCNegCtrlEn_flg] -> Unit Delay23/1
  [VVMC_ZCPosDetEn_flg] -> Unit Delay30/1
  Constant188/1 -> Relational Operator100/2
  Unit Delay30/1 -> AND44/1, AND42/3
  Constant189/1 -> AND42/1
  Relational Operator100/1 -> AND42/2
  Constant190/1 -> NOT23/1
  [VVMC_TotalRealWhlTq_Nm] -> Relational Operator100/1
  NOT23/1 -> AND44/2
  AND42/1 -> AND43/1
  AND44/1 -> AND43/2
  AND47/1 -> AND46/2
  AND45/1 -> AND46/1
  NOT24/1 -> AND47/2
  [VVMC_TotalRealWhlTq_Nm] -> Relational Operator101/1
  Constant194/1 -> NOT24/1
  Relational Operator101/1 -> AND45/2
  Constant193/1 -> AND45/1
  Unit Delay22/1 -> AND45/3, AND47/1
  Constant191/1 -> Relational Operator101/2
  [VVMC_ZCPosCtrlEn_flg] -> Unit Delay22/1
  [VINP_FrEDURotateDirction_enum] -> Terminator/1
  Constant196/1 -> Relational Operator69/2
  [VINP_RrEDURotateDirction_enum] -> Relational Operator69/1
  Relational Operator69/1 -> AND33/1
  Constant148/1 -> AND33/2
  AND33/1 -> OR13/2
  Constant160/1 -> AND48/2
  Relational Operator86/1 -> AND48/1
  [VINP_RrEDURotateDirction_enum] -> Relational Operator86/1
  Constant195/1 -> Relational Operator86/2
  OR16/1 -> Switch63/2
  AND48/1 -> OR16/2
  [VVMC_ZeroSpdTMSpdCtrlTarget_rpm] -> Relational Operator85/1
  Constant155/1 -> Relational Operator85/2
  Relational Operator85/1 -> NOT25/1
  NOT25/1 -> Detect Increase5/1
  Detect Increase5/1 -> Switch57/2
  Switch59/1 -> Switch57/1
  [VINP_RRWhlRotDir_enum] -> Relational Operator90/1
  [VINP_LRWhlRotDir_enum] -> Relational Operator87/1
  Constant165/1 -> Relational Operator87/2
  Constant170/1 -> Relational Operator90/2
  OR17/1 -> Switch59/2
  Relational Operator87/1 -> OR17/1
  Relational Operator90/1 -> OR17/2
  Constant169/1 -> Switch59/1
  Switch61/1 -> Switch59/3
  Relational Operator94/1 -> OR18/2
  Relational Operator91/1 -> OR18/1
  Constant177/1 -> Relational Operator94/2
  Constant175/1 -> Relational Operator91/2
  [VINP_LRWhlRotDir_enum] -> Relational Operator91/1
  [VINP_RRWhlRotDir_enum] -> Relational Operator94/1
  OR18/1 -> Switch61/2
  Constant178/1 -> Switch61/1
  Constant183/1 -> Switch61/3
  Switch57/1 -> Unit Delay24/1, Cast To Single1/1
  Unit Delay24/1 -> [VVMC_LastWhlDir4JP_enum]
  Switch64/1 -> Switch57/3
  [VVMC_LastWhlDir4JP_enum] -> Relational Operator95/1
  Constant184/1 -> Relational Operator95/2
  Relational Operator95/1 -> Switch64/2
  Relational Operator97/1 -> OR15/2
  Relational Operator96/1 -> OR15/1
  Constant186/1 -> Relational Operator97/2
  Constant185/1 -> Relational Operator96/2
  [VINP_LRWhlRotDir_enum] -> Relational Operator96/1
  [VINP_RRWhlRotDir_enum] -> Relational Operator97/1
  OR19/1 -> [VVMC_RrWhlStandstill_flg]  "VVMC_RrWhlStandstill_flg"
  [VVMC_RrWhlStandstill_flg] -> Switch65/2
  Constant187/1 -> Switch65/1
  Switch69/1 -> Switch68/3, Switch67/3, Switch65/3
  Switch65/1 -> Switch64/1
  Switch67/1 -> Switch66/1
  Constant198/1 -> Switch67/1
  [VVMC_RrWhlStandstill_flg] -> Switch67/2
  Relational Operator102/1 -> Switch66/2
  Constant197/1 -> Relational Operator102/2
  [VVMC_LastWhlDir4JP_enum] -> Relational Operator102/1
  Switch66/1 -> Switch64/3
  [VINP_RrEDURotateDirction_enum] -> Relational Operator103/1
  Relational Operator103/1 -> AND49/1
  Constant202/1 -> Relational Operator103/2
  Constant201/1 -> AND49/2
  OR15/1 -> OR19/2
  AND49/1 -> OR19/1
  Switch68/1 -> Switch66/3
  [VVMC_RrWhlStandstill_flg] -> Switch68/2
  Constant200/1 -> Switch68/1
  Constant204/1 -> Switch69/1
  Relational Operator105/1 -> OR20/2
  Relational Operator104/1 -> OR20/1
  OR20/1 -> Switch69/2
  Constant205/1 -> Relational Operator105/2
  Constant203/1 -> Relational Operator104/2
  [VINP_LRWhlRotDir_enum] -> Relational Operator104/1
  [VINP_RRWhlRotDir_enum] -> Relational Operator105/1
  Constant206/1 -> Switch69/3
  [VVMC_RrWhlStandstill_flg] -> VVMC_RrWhlStandstill_flg/1
  [VVMC_ACCVehHoldReqRaw_flg] -> OR2/3
  [VVMC_ACCVehHoldReqRaw_flg] -> OR11/3
  [VVMC_ACCDeltaTqGradeGn_Nm] -> Relational Operator106/1
  Constant192/1 -> Relational Operator106/2
  AND50/1 -> Switch70/2
  Relational Operator106/1 -> AND50/1
  Constant199/1 -> AND50/2
  Switch78/1 -> [VVMC_HoldTqGradeGnFinal_Nm], Switch74/1  "VVMC_HoldTqGradeGnFinal_Nm"
  Switch74/1 -> Min9/2
  Switch76/1 -> Switch70/3
  [VVMC_OriADASWhlTq_Nm] -> Min9/1
  Min9/1 -> Switch79/3
  Switch70/1 -> Switch50/1
  Unit Delay32/1 -> Min10/1
  [VVMC_EstSlope_Deg] -> Switch71/3
  [VVMC_ACCVehHoldReqRaw_flg] -> Switch71/2
  [VVMC_EstSlope_Deg] -> Relational Operator117/1
  Min10/1 -> Switch72/1
  [VVMC_VehicleSpeed_kph] -> Relational Operator107/1
  Constant207/1 -> Relational Operator107/2
  Constant208/1 -> Relational Operator108/2
  [VINP_MCPressure_bar] -> Relational Operator108/1
  Relational Operator108/1 -> AND34/3
  [VVMC_VehicleSpeed_kph] -> Relational Operator109/1
  Constant209/1 -> Relational Operator109/2
  Relational Operator109/1 -> AND51/3
  Detect Increase6/1 -> Triggered Subsystem5/Trigger
  [VVMC_LastADASWhlTqCal_Nm] -> Triggered Subsystem5/1(In1)
  [VVMC_LongAcc_Gps] -> Triggered Subsystem5/2(In2)
  Triggered Subsystem5/1(Out1) -> [VVMC_HoldTqCalSpd1Tq_Nm]  "VVMC_HoldTqCalSpd1Tq_Nm"
  Triggered Subsystem5/2(Out2) -> [VVMC_HoldTqCalSpd1Gx_Gps]  "VVMC_HoldTqCalSpd1Gx_Gps"
  [VVMC_ACCVehHoldReqRaw_flg] -> NOT26/1
  NOT26/1 -> AND51/2
  AND51/1 -> SR_Latch15/1
  [VVMC_ACCVehHoldReqRaw_flg] -> AND54/3
  AND54/1 -> Detect Increase7/1
  Detect Increase7/1 -> SR_Latch14/1, Triggered Subsystem6/Trigger
  [VVMC_LastADASWhlTqCal_Nm] -> Triggered Subsystem6/1(In1)
  [VVMC_LongAcc_Gps] -> Triggered Subsystem6/2(In2)
  [VVMC_HoldTqCalSpd1Det_flg] -> AND54/1
  NOT28/1 -> AND54/2
  [VVMC_AccelTurnHold_flg] -> NOT28/1
  SR_Latch14/1 -> [VVMC_HoldTqCalEn_flg]  "VVMC_HoldTqCalEn_flg"
  [VVMC_ACCVehHoldReqRaw_flg] -> NOT29/1
  NOT29/1 -> SR_Latch14/2
  Triggered Subsystem6/1(Out1) -> [VVMC_HoldTqCalSpd2Tq_Nm]  "VVMC_HoldTqCalSpd2Tq_Nm"
  Triggered Subsystem6/2(Out2) -> [VVMC_HoldTqCalSpd2Gx_Gps]  "VVMC_HoldTqCalSpd2Gx_Gps"
  [VVMC_HoldTqCalSpd1Tq_Nm] -> Add32/2
  [VVMC_HoldTqCalSpd2Tq_Nm] -> Add32/1
  [VVMC_HoldTqCalSpd2Gx_Gps] -> Add33/1
  [VVMC_HoldTqCalSpd1Gx_Gps] -> Add33/2
  Abs/1 -> Relational Operator111/1
  Add33/1 -> Abs/1
  Constant212/1 -> Relational Operator111/2
  Relational Operator111/1 -> AND53/1
  [VVMC_HoldTqCalEn_flg] -> AND53/2
  AND53/1 -> [VVMC_HoldTqCtrlEn_flg]  "VVMC_HoldTqCtrlEn_flg"
  Add32/1 -> divide/1
  [VVMC_HoldTqCalSpd1Gx_Gps] -> Add34/2
  [VVMC_HoldTqCalSpd2Gx_Gps] -> Add34/1
  Add34/1 -> divide/2
  Constant213/1 -> divide/3
  divide/1 -> [VVMC_HoldTqGxRat_raw32]  "VVMC_HoldTqGxRat_raw32"
  Constant214/1 -> Product2/1
  [VVMC_HoldTqCalSpd2Gx_Gps] -> Add35/2
  Add35/1 -> Product3/1
  [VVMC_HoldTqGxRat_raw32] -> Product3/2
  [VVMC_HoldTqCalSpd2Tq_Nm] -> Add36/1
  Add36/1 -> [VVMC_HoldTqTarget_Nm]  "VVMC_HoldTqTarget_Nm"
  Product3/1 -> Add36/2
  Constant215/1 -> Switch73/3
  AND55/1 -> Switch73/2
  [VVMC_HoldTqTarget_Nm] -> Switch73/1
  [VVMC_HoldTqCtrlEn_flg] -> AND55/1
  Constant216/1 -> AND55/2
  Switch73/1 -> [VVMC_HoldTqTargetFinal_Nm]  "VVMC_HoldTqTargetFinal_Nm"
  [VVMC_HoldTqTargetFinal_Nm] -> Min11/2
  [VVMC_ACCDeltaTqGradeGn_Nm] -> Min11/1
  Constant217/1 -> Switch74/2
  Min14/1 -> Switch74/3
  Constant218/1 -> AND57/1
  MVMC_VHTMSpdCtrl_Z_Nm/1 -> Min12/2, Switch75/3
  Switch77/1 -> Add39/2
  [VVMC_LastADASWhlTqCal_Nm] -> Relational Operator110/2
  [task_time_s] -> Divide4/2
  [VVMC_UphillTqIncSR_Nm] -> Divide11/1
  Constant220/1 -> Divide11/2
  Add38/1 -> Min14/2
  [VVMC_LastADASWhlTqCal_Nm] -> Add38/1
  [VVMC_UphillTqIncSR_Nm] -> Add38/2
  [VVMC_ACCDeltaTqGradeGn_Nm] -> Min14/1
  Min11/1 -> Relational Operator110/1
  [VVMC_AccelTurnHold_flg] -> NOT30/1
  NOT30/1 -> AND50/3
  AND56/1 -> Switch76/2
  [VVMC_OriADASWhlTq_Nm] -> Switch76/3
  Constant223/1 -> AND56/2
  Relational Operator112/1 -> AND56/1
  Constant219/1 -> Relational Operator112/2
  [VVMC_ACCDeltaTqGradeGn_Nm] -> Relational Operator112/1
  [VVMC_AccelTurnHold_flg] -> AND56/3
  [VVMC_AccelTurnHold_flg] -> Switch77/2
  Constant222/1 -> Divide4/1
  Divide11/1 -> Switch77/3
  [VVMC_OriADASWhlTq_Nm] -> Min8/2
  Min8/1 -> Switch76/1
  [VVMC_HoldTqGradeGnFinal_Nm] -> Min8/1
  [VVMC_LastADASWhlTqCal_Nm] -> Add31/2
  Add31/1 -> Min12/1
  [VVMC_HoldTqGradeGnFinal_Nm] -> Add31/1
  Min12/1 -> Switch75/1
  Constant221/1 -> Relational Operator113/2
  [VVMC_ACCDeltaTqGradeGn_Nm] -> Relational Operator113/1
  AND57/1 -> Switch75/2
  Relational Operator113/1 -> AND57/2
  Constant210/1 -> Product2/2
  Product2/1 -> Add35/1
  Constant224/1 -> Relational Operator114/2
  [VVMC_ADASACCSta_enum] -> Relational Operator114/1
  Relational Operator114/1 -> AND51/1
  SR_Latch15/1 -> [VVMC_HoldTqCalSpd1Det_flg], Detect Increase6/1  "VVMC_HoldTqCalSpd1Det_flg"
  [VVMC_VehicleSpeed_kph] -> Relational Operator115/1
  Constant225/1 -> Relational Operator115/2
  [VVMC_ADASACCSta_enum] -> Relational Operator116/1
  Constant226/1 -> Relational Operator116/2
  Relational Operator115/1 -> AND58/1
  Relational Operator116/1 -> AND58/3
  AND58/1 -> SR_Latch15/2
  [VVMC_ACCVehHoldReqRaw_flg] -> Unit Delay33/1
  Unit Delay33/1 -> AND58/2
  Relational Operator110/1 -> Switch78/2
  [VVMC_UphillTqIncSR_Nm] -> Add37/2
  [VVMC_LastADASWhlTqCal_Nm] -> Add37/1
  Add37/1 -> Min13/2
  Min13/1 -> Switch78/1
  [VVMC_ACCDeltaTqGradeGn_Nm] -> Min15/1
  [VVMC_HoldTqTargetFinal_Nm] -> Min15/2
  Min15/1 -> Min13/1
  Min17/1 -> Min16/1
  [VVMC_HoldTqTargetFinal_Nm] -> Min17/2
  [VVMC_ACCDeltaTqGradeGn_Nm] -> Min17/1
  Add39/1 -> Min16/2
  [VVMC_LastADASWhlTqCal_Nm] -> Add39/1
  Min16/1 -> Switch78/3
  Divide4/1 -> Switch77/1
  Switch72/1 -> Unit Delay32/1, Switch71/1
  [VVMC_ACCVehHoldReq_flg] -> Detect Decrease/1
  [VVMC_ADASACCSta_enum] -> Relational Operator118/1
  Constant211/1 -> Relational Operator118/2
  [VVMC_VehicleSpeed_kph] -> Relational Operator119/1
  Constant231/1 -> Relational Operator119/2
  Constant232/1 -> Relational Operator120/2
  [VVMC_ADASACCSta_enum] -> Relational Operator120/1
  AND52/1 -> SR_Latch8/1
  Relational Operator118/1 -> AND52/2
  Detect Decrease/1 -> AND52/1
  Relational Operator120/1 -> AND59/3
  Relational Operator119/1 -> AND59/1
  AND59/1 -> SR_Latch8/2
  [VVMC_ACCVehHoldReqRaw_flg] -> AND59/2
  SR_Latch8/1 -> [VVMC_HoldResTqEn_flg]  "VVMC_HoldResTqEn_flg"
  [VVMC_ActAccDev_mps2] -> Relational Operator121/1
  Constant233/1 -> Relational Operator121/2
  Relational Operator121/1 -> AND59/4
  [VVMC_HoldResTqEn_flg] -> Switch84/2
  Constant234/1 -> Switch84/3
  Switch84/1 -> [VVMC_HoldResTq_Nm]  "VVMC_HoldResTq_Nm"
  MVMC_HoldResTq_Y_Nm/1 -> Switch84/1
  [VVMC_VehicleSpeed_kph] -> MVMC_HoldResTq_Y_Nm/1
  [VVMC_HoldResTq_Nm] -> Add1/5
  VVMC_ACCVehHoldReq_flg/1 -> [VVMC_ACCVehHoldReq_flg]
  Constant228/1 -> Relational Operator117/2
  Relational Operator117/1 -> AND60/1
  Constant227/1 -> AND60/2
  AND60/1 -> Switch72/2
  [VVMC_EstSlope_Deg] -> Min10/2
  [VVMC_EstSlope_Deg] -> Switch72/3
  [VVMC_LongAcc_Gps] -> Product4/1
  Constant229/1 -> Product4/2
  Product4/1 -> Relational Operator122/1, Detect Increase8/1
  Constant230/1 -> Relational Operator122/2
  AND61/1 -> SR_Latch16/1
  Detect Increase8/1 -> AND61/2
  Relational Operator122/1 -> AND61/3
  [VVMC_ACCVehHoldReqRaw_flg] -> AND61/1
  [VVMC_ACCVehHoldReq_flg] -> NOT27/1
  NOT27/1 -> AND62/1
  SR_Latch16/1 -> [VVMC_HoldTqAddDis_flg]  "VVMC_HoldTqAddDis_flg"
  Switch79/1 -> Switch70/1, Unit Delay31/1
  [VVMC_HoldTqAddDis_flg] -> Switch79/2
  Switch80/1 -> Switch79/1
  [VVMC_HoldTqAddDis_flg] -> NOT31/1
  NOT31/1 -> AND57/3
  VVMC_ACCShutOffHold_flg/1 -> [VVMC_ACCShutOffHold_flg]
  [VVMC_ACCShutOffHold_flg] -> NOT32/1
  NOT32/1 -> OR5/3
  [VVMC_ACCVehHoldReqRaw_flg] -> NOT33/1
  AND62/1 -> SR_Latch16/2
  NOT33/1 -> AND62/2
  Constant235/1 -> Relational Operator123/2
  [VINP_MCPressure_bar] -> Relational Operator123/1
  Relational Operator123/1 -> Switch80/2
  [VVMC_OriADASWhlTq_Nm] -> Switch80/1
  Unit Delay31/1 -> [VVMC_Last1stHoldTq_Nm]
  [VVMC_Last1stHoldTq_Nm] -> Switch80/3
  [VINP_RFWhlRotDir_enum] -> Terminator1/1
  [VINP_LFWhlRotDir_enum] -> Terminator2/1
  VVMC_RrWhlSpdInvalid_flg/1 -> [VVMC_RrWhlSpdInvalid_flg]
  VVMC_LongAccFrWhl_Gps/1 -> [VVMC_LongAccFrWhl_Gps]
  VVMC_FrWhlSpdInvalid_flg/1 -> [VVMC_FrWhlSpdInvalid_flg]
  VVMC_LongAccRrWhl_Gps/1 -> [VVMC_LongAccRrWhl_Gps]
  Constant236/1 -> Switch81/2
  Add7/1 -> Switch81/3
  [VVMC_ACCDeltaAclAftCompare_mps2] -> Switch81/1
  [VVMC_FrWhlSpdInvalid_flg] -> OR21/1
  Add40/1 -> Switch82/1
  [VVMC_FrWhlSpdInvalid_flg] -> Switch83/2
  [VVMC_LongAcc_Gps] -> Product5/1
  Product5/1 -> Add40/2
  Constant237/1 -> Product5/2
  [VVMC_ACCReqAclAftLim_mps2] -> Add40/1
  [VVMC_RrWhlSpdInvalid_flg] -> OR21/2
  OR21/1 -> Switch82/2
  Switch83/1 -> Switch82/3
  Switch85/1 -> Switch83/3
  [VVMC_RrWhlSpdInvalid_flg] -> Switch85/2
  [VVMC_ACCReqAclAftLim_mps2] -> Add41/1
  Constant238/1 -> Product6/2
  Product6/1 -> Add41/2
  [VVMC_LongAcc_Gps] -> Product6/1
  [VVMC_ACCReqAclAftLim_mps2] -> Add43/1
  Constant240/1 -> Product8/2
  Product8/1 -> Add43/2
  [VVMC_LongAccRrWhl_Gps] -> Product8/1
  Add41/1 -> Switch86/1, Abs1/1
  Add43/1 -> Switch86/3, Abs2/1
  Abs1/1 -> Relational Operator124/1
  Abs2/1 -> Relational Operator124/2
  Relational Operator124/1 -> Switch86/2
  Switch86/1 -> Switch83/1
  Relational Operator125/1 -> Switch87/2
  Abs4/1 -> Relational Operator125/2
  Abs3/1 -> Relational Operator125/1
  Add45/1 -> Abs4/1, Switch87/3
  Add44/1 -> Abs3/1, Switch87/1
  [VVMC_LongAccFrWhl_Gps] -> Product10/1
  Product10/1 -> Add45/2
  Constant242/1 -> Product10/2
  [VVMC_ACCReqAclAftLim_mps2] -> Add45/1
  [VVMC_LongAcc_Gps] -> Product9/1
  Product9/1 -> Add44/2
  Constant241/1 -> Product9/2
  [VVMC_ACCReqAclAftLim_mps2] -> Add44/1
  Switch87/1 -> Switch85/1
  Relational Operator126/1 -> Switch88/2
  Abs6/1 -> Relational Operator126/2
  Abs5/1 -> Relational Operator126/1
  Add46/1 -> Abs6/1, Switch88/3
  Add42/1 -> Abs5/1, Switch88/1
  [VVMC_LongAccRrWhl_Gps] -> Product11/1
  Product11/1 -> Add46/2
  Constant243/1 -> Product11/2
  [VVMC_ACCReqAclAftLim_mps2] -> Add46/1
  [VVMC_LongAcc_Gps] -> Product7/1
  Product7/1 -> Add42/2
  Constant239/1 -> Product7/2
  [VVMC_ACCReqAclAftLim_mps2] -> Add42/1
  Switch88/1 -> Switch89/1, Abs7/1
  [VVMC_ACCReqAclAftLim_mps2] -> Add48/1
  Constant245/1 -> Product12/2
  Product12/1 -> Add48/2
  [VVMC_LongAccFrWhl_Gps] -> Product12/1
  Add48/1 -> Switch89/3, Abs8/1
  Abs7/1 -> Relational Operator127/1
  Abs8/1 -> Relational Operator127/2
  Relational Operator127/1 -> Switch89/2
  Switch89/1 -> Switch85/3
  Switch82/1 -> [VVMC_ACCDeltaAclAftCompare_mps2]  "VVMC_ACCDeltaAclAftCompare_mps2"
